simulink model "MIL4L3_SW6_V1_20220211"  (R2018b)
settings: Solver=FixedStepAuto  StartTime=0.0  StopTime=inf  FixedStep=0.001  RelTol=1e-3
PreLoadFcn:
  | A0_MILtest;
undefined symbols (not defined in the file or in its folder): Clb_ICADirect_LaneDisp_StateFive, Clb_ICADirect_LaneDisp_StateFour, Clb_ICADirect_LaneDisp_StateOne, Clb_ICADirect_LaneDisp_StateThree, Clb_ICADirect_LaneDisp_StateTwo, Clb_ICADirect_LaneDisp_StateZero, Clb_ICADirect_LaneDispSW, Clb_ICADirect_TrnLghtsCom_Switch, Clb_ICADirect_TrnLghtsCom_Value, Clb_ICADirect_TrnLghtsCrtl_Inhb, IMAP_Clb_ACU_Driver_Belt, IMAP_Clb_ACU_Driver_Belt_Over, IMAP_Clb_ACU_Passenger_Belt, IMAP_Clb_ACU_Passenger_Belt_Over, IMAP_Clb_ACU_RearLeft_Belt, IMAP_Clb_ACU_RearLeft_Belt_Over, IMAP_Clb_ACU_RearMiddle_Belt, IMAP_Clb_ACU_RearMiddle_Belt_Over, IMAP_Clb_ACU_RearRight_Belt, IMAP_Clb_ACU_RearRight_Belt_Over, IMAP_Clb_AEB_Switch, IMAP_Clb_AEB_Switch_Over, IMAP_Clb_ALC_TLC_Mode, IMAP_Clb_ALC_TLC_Mode_Over, IMAP_Clb_BCM_Battery_Voltage, IMAP_Clb_BCM_Battery_Voltage_Over, IMAP_Clb_BCM_BrakeLamp_State, IMAP_Clb_BCM_BrakeLamp_State_Over, IMAP_Clb_BCM_CHMSL_Status, IMAP_Clb_BCM_CHMSL_Status_Over, IMAP_Clb_BCM_Door_Lock_State, IMAP_Clb_BCM_Door_Lock_State_Over, IMAP_Clb_BCM_FrontWiper_State, IMAP_Clb_BCM_FrontWiper_State_Over, IMAP_Clb_BCM_FrontWiper_Switch, IMAP_Clb_BCM_FrontWiper_Switch_Over, IMAP_Clb_BCM_HazardLamp, IMAP_Clb_BCM_HazardLamp_Over, IMAP_Clb_BCM_HazardLamp_Switch, IMAP_Clb_BCM_HazardLamp_Switch_Over, IMAP_Clb_BCM_HighBeam_State, IMAP_Clb_BCM_HighBeam_State_Over, IMAP_Clb_BCM_Ignition_State, IMAP_Clb_BCM_Ignition_State_Over, IMAP_Clb_BCM_IHBC_Enabled, IMAP_Clb_BCM_IHBC_Enabled_Over, IMAP_Clb_BCM_Left_Light, IMAP_Clb_BCM_Left_Light_Over, IMAP_Clb_BCM_LeftTurn_Switch, IMAP_Clb_BCM_LeftTurn_Switch_Over, IMAP_Clb_BCM_LF_Door_State, IMAP_Clb_BCM_LF_Door_State_Over, IMAP_Clb_BCM_LowBeam_State, IMAP_Clb_BCM_LowBeam_State_Over, IMAP_Clb_BCM_LR_Door_State, IMAP_Clb_BCM_LR_Door_State_Over, IMAP_Clb_BCM_RF_Door_State, IMAP_Clb_BCM_RF_Door_State_Over, IMAP_Clb_BCM_Right_Light, IMAP_Clb_BCM_Right_Light_Over ... (+547)
libraries: CarMaker4SL x2153, simulink x292, dspstat3 x3, canmsglib x2, simulink_extras x1
(part 6 of 52)

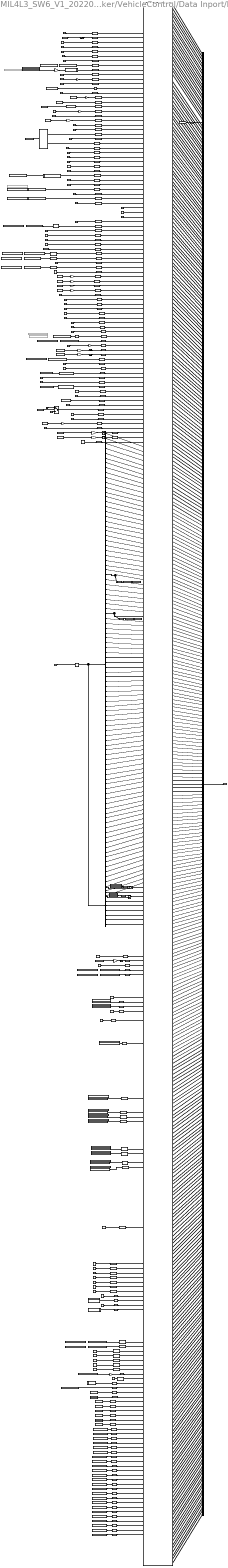
== system MIL4L3_SW6_V1_20220211/CarMaker/VehicleControl/Data Inport/IMAP ==
  note: 根据ACC反馈更新
  note: 需要补充输入数据
  note: 根据规控反馈，由0改为1
  note: 2是打开FAPA
      | else是关闭FAPA
  note: 单位转换：Bar-MPa
  note: 0:无故障
      | 1:故障
  note: 制动轮缸压力
  note: 0：无输入
      | 1：MP5不工作
      | 2：MP5工作
      | 3：无效
  note: 0： Reserved
      | 1： ISA
      | 2： ISLC
      | 3： Reserved
  note: 0：ESA OFF
      | 1：ESA ON
      | 2：Reserved
      | 3： Reserved
  note: 0：Single Lane（ICA）（default）
      | 1：ICAReserved
      | 2：TLC
      | 3：ALC+TLC
  note: 根据规控反馈，由0改为1
  note: 根据acc反馈补充
  note: 0:Available
      | 1:Not available
  note: 0：自适应巡航（ACC）
      | 1：智能领航（ICA）
      | 2：Reserved
      | 3： Reserved
  SDFA_L3- : Inport
  1 : CarMaker4SL/Read CM Dict  xname=Car.vFL  xsync=off
  2 : CarMaker4SL/Read CM Dict  xname=Car.vFR  xsync=off
  3 : CarMaker4SL/Read CM Dict  xname=Car.vRL  xsync=off
  4 : CarMaker4SL/Read CM Dict  xname=Car.vRR  xsync=off
  ACCEL_LONGI_CALIB1 : Saturate  UpperLimit=40.92  LowerLimit=-40.96
  ACU_DriverBeltSwitchSig : Constant  Value=0
  ACU_PassengerBeltSwitchSig : Constant  Value=0
  BCM_BrakeLampStatus : Constant  Value=0
  BCM_CHMSLStatus : Constant  Value=0
  BCM_FrontWiperWorkSt : Constant  Value=0
  BCM_HazardSwitchSt : Constant  Value=0  OutDataTypeStr=uint8
  BCM_HighBeamStatus : Constant  Value=0
  BCM_IgnitionSt : Constant  Value=2
  Bus Selector : BusSelector  OutputSignals=SDFAve_y_ISAValue (signal 28),SDFAve_y_ISAPopupMessage (signal 88),SDFAve_y_ISASignType (signal 86),SDFAve_y_ISAStatus (signal 87),SDFAve_y_TSR_Sign_Type (signal 29),SDFAve_g_CameraSignalFault (signal 30),SDFAve_y_Radar_State (signal 89),SDFAve_y_OperatinfStatus (signal 90),SDFAve_y_Radar_FaultBitSetting_Signal (signal 94)
  Bus Selector1 : BusSelector  OutputSignals=SDFAve_d_sensor_status (signal 1),SDFAve_d_sen_sta_LF_radar (signal 2),SDFAve_d_sen_sta_RF_radar (signal 3),SDFAve_d_sen_sta_LB_radar (signal 4),SDFAve_d_sen_sta_RB_radar (signal 5),SDFAve_d_fusion_status (signal 6),SDFAve_g_fusion_time_stamp (signal 7),SDFAve_d_obj_Num (signal 8),SDFAva_d_obj_id (signal 9),SDFAva_g_obj_pos_x (signal 10),SDFAva_g_obj_pos_y (signal 11),SDFAva_g_obj_vel_x (signal 12),SDFAva_g_obj_vel_y (signal 13),SDFAva_g_obj_acc_x (signal 14),SDFAva_g_obj_acc_y (signal 15),SDFAva_g_obj_pos_var_x (signal 16),SDFAva_g_obj_pos_var_y (signal 17),SDFAva_g_obj_pos_var_xy (signal 18),SDFAva_g_obj_width (signal 19),SDFAva_g_obj_length (signal 20),SDFAva_d_obj_class (signal 21),SDFAva_d_obj_lane (signal 22),SDFAva_y_obj_status (signal 23),SDFAve_g_obj_age (signal 24),SDFAva_y_obj_TurnLight (signal 25),SDFAva_d_obj_BrakeLight (signal 26),SDFAva_y_obj_MotionStatus (signal 27),SDFAve_y_Road_TYPE (signal 31),SDFAve_g_L0_C0_COEF (signal 32),SDFAve_g_L0_C1_COEF (signal 33),SDFAve_g_L0_C2_COEF (signal 34),SDFAve_g_L0_C3_COEF (signal 35),SDFAve_g_L0_VIEW_RANGE (signal 36),SDFAve_g_L0_DETECT_QUALITY (signal 37),SDFAve_d_L0_LINE_TYPE (signal 38),SDFAve_g_L0_MARK_WIDTH (signal 39),SDFAve_g_R0_C0_COEF (signal 40),SDFAve_g_R0_C1_COEF (signal 41),SDFAve_g_R0_C2_COEF (signal 42),SDFAve_g_R0_C3_COEF (signal 43),SDFAve_g_R0_VIEW_RANGE (signal 44),SDFAve_y_R0_DETECT_QUALITY (signal 45),SDFAve_d_R0_LINE_TYPE (signal 46),SDFAve_g_R0_MARK_WIDTH (signal 47),SDFAve_g_R0_VIEW_RANGE (signal 48),SDFAve_g_L1_C1_COEF (signal 49),SDFAve_g_L1_C2_COEF (signal 50),SDFAve_g_L1_C3_COEF (signal 51),SDFAve_g_L1_VIEW_RANGE (signal 52),SDFAve_y_L1_DETECT_QUALITY (signal 53),SDFAve_d_L1_LINE_TYPE (signal 54),SDFAve_g_L1_MARK_WIDTH (signal 55),SDFAve_g_R1_C0_COEF (signal 56),SDFAve_g_R1_C1_COEF (signal 57),SDFAve_g_R1_C2_COEF (signal 58),SDFAve_g_R1_C3_COEF (signal 59),SDFAve_g_R1_VIEW_RANGE (signal 60),SDFAve_y_R1_DETECT_QUALITY (signal 61),SDFAve_d_R1_LINE_TYPE (signal 62),SDFAve_g_R1_MARK_WIDTH (signal 63),SDFAve_g_L0_C0_BACK_COEF (signal 64),SDFAve_g_L0_C1_BACK_COEF (signal 65),SDFAve_g_L0_C2_BACK_COEF (signal 66),SDFAve_g_L0_C3_BACK_COEF (signal 67),SDFAve_g_L0_BACK_RANGE (signal 68),SDFAve_g_R0_C0_BACK_COEF (signal 69),SDFAve_g_R0_C1_BACK_COEF (signal 70),SDFAve_g_L0_C0_BACK_COEF (signal 71),SDFAve_g_R0_C3_BACK_COEF (signal 72),SDFAve_g_R0_BACK_RANGE (signal 73),SDFAve_g_L1_C0_BACK_COEF (signal 74),SDFAve_g_L1_C1_BACK_COEF (signal 75),SDFAve_g_L1_C2_BACK_COEF (signal 76),SDFAve_g_L1_C3_BACK_COEF (signal 77),SDFAve_g_L1_BACK_RANGE (signal 78),SDFAve_g_R1_C0_BACK_COEF (signal 79),SDFAve_g_R1_C1_BACK_COEF (signal 80),SDFAve_g_R1_C2_BACK_COEF (signal 81),SDFAve_g_R1_C3_BACK_COEF (signal 82),SDFAve_g_R1_BACK_RANGE (signal 83),SDFAve_g_Lrg_C0_BACK_COEF (signal 95),SDFAve_g_Lrg_C1_BACK_COEF (signal 96),SDFAve_g_Lrg_C2_BACK_COEF (signal 97),SDFAve_g_Lrg_C3_BACK_COEF (signal 98),SDFAve_g_Lrg_VIEW_RANGE_start (signal 99),SDFAve_g_Lrg_VIEW_RANGE_end (signal 100),SDFAve_y_Lrg_DETECT_QUALITY (signal 109),SDFAve_y_Lrg_LINE_TYPE (signal 110),SDFAve_g_Rrg_C0_BACK_COEF (signal 101),SDFAve_g_Rrg_C1_BACK_COEF (signal 102),SDFAve_g_Rrg_C2_BACK_COEF (signal 103),SDFAve_g_Rrg_C3_BACK_COEF (signal 104),SDFAve_g_Rrg_VIEW_RANGE_start (signal 105),SDFAve_g_Rrg_VIEW_RANGE_end (signal 106),SDFAve_y_Rrg_DETECT_QUALITY (signal 107),SDFAve_y_Rrg_LINE_TYPE (signal 108)
  BusCreator : BusCreator  Inputs=425
  CIPV_ID1 : Subsystem
  Compare To Constant2 : simulink/Logic and Bit Operations/Compare To Constant  relop=>=  const=0.5  OutDataTypeStr=boolean
  Constant{1..2,15,20,22,24..27} (9 alike) : Constant  Value=0
  Constant10 : Constant
  Constant18 : Constant
  Constant19 : Constant
  Constant21 : Constant  Value=2
  Constant23 : Constant  Value=0  OutDataTypeStr=uint8
  Data Type  Conversion{1..16,19..22,24..27,32,36..37,41..42,44..52,54..58,60,63..64,71..73,75..83,86..87,89..96,98..99,101,103..106,108..110,112..113,115,131..134,141,149,156,158..159,162,171,290,292..295,297} (98 alike) : DataTypeConversion
  Data Type  Conversion180 : DataTypeConversion  OutDataTypeStr=UInt16
  Data Type Conversion{,1..13,21..43,46..47,51..54,56,58..59,61,64..65,67,72..73,92,211..212,216,223..227,230,238..241,244,246} (68 alike) : DataTypeConversion
  Data Type Conversion48 : DataTypeConversion  OutDataTypeStr=T_M_Nm_Float32
  Data Type Conversion49 : DataTypeConversion  OutDataTypeStr=T_M_Nm_Float32
  Define CM Dict : CarMaker4SL/Define CM Dict  xname=User.IO.Out.R0_C1  xmono=off  xtype=Double4  xdvaplace=None  xnstates=0  xfirststate=0  xinitial=0
  Define CM Dict1 : CarMaker4SL/Define CM Dict  xname=User.IO.Out.EPS_LKAState  xmono=off  xtype=Double4  xdvaplace=IO_Out  xnstates=0  xfirststate=0  xinitial=0
  Define CM Dict10 : CarMaker4SL/Define CM Dict  xname=User.IO.Out.ISA_SignType  xmono=off  xtype=Double4  xdvaplace=IO_Out  xnstates=0  xfirststate=0  xinitial=0
  Define CM Dict11 : CarMaker4SL/Define CM Dict  xname=User.IO.Out.BCM_LeftTurnSwitchSt  xunit=Nm  xmono=off  xtype=Double4  xdvaplace=IO_Out  xnstates=0  xfirststate=0  xinitial=0
  Define CM Dict12 : CarMaker4SL/Define CM Dict  xname=User.IO.Out.BCM_RightTurnSwicthSt  xunit=Nm  xmono=off  xtype=Double4  xdvaplace=IO_Out  xnstates=0  xfirststate=0  xinitial=0
  Define CM Dict15 : CarMaker4SL/Define CM Dict  Commented=on  xname=User.IO.Out.Brake_pedal_position  xunit=%  xmono=off  xtype=Double4  xdvaplace=IO_Out  xnstates=0  xfirststate=0  xinitial=0
  Define CM Dict17 : CarMaker4SL/Define CM Dict  xname=User.IO.Out.Mp5TLCMode  xunit=Nm  xmono=off  xtype=Double4  xdvaplace=IO_Out  xnstates=0  xfirststate=0  xinitial=0
  Define CM Dict2 : CarMaker4SL/Define CM Dict  xname=User.IO.Out.BCM_HazardLampSt  xmono=off  xtype=Double4  xdvaplace=IO_Out  xnstates=0  xfirststate=0  xinitial=0
  Define CM Dict22 : CarMaker4SL/Define CM Dict  xname=User.IO.Out.EPS_ESAState  xmono=off  xtype=Double4  xdvaplace=IO_Out  xnstates=0  xfirststate=0  xinitial=0
  Define CM Dict27 : CarMaker4SL/Define CM Dict  xname=User.IO.Out.MP5_JA_Modes  xunit=Nm  xmono=off  xtype=Double4  xdvaplace=IO_Out  xnstates=0  xfirststate=0  xinitial=0
  Define CM Dict28 : CarMaker4SL/Define CM Dict  xname=User.IO.Out.MP5_JA_Alert_Switch  xunit=Nm  xmono=off  xtype=Double4  xdvaplace=IO_Out  xnstates=0  xfirststate=0  xinitial=0
  Define CM Dict29 : CarMaker4SL/Define CM Dict  xname=User.IO.Out.MP5_AutoPilotSwitch  xmono=off  xtype=Double4  xdvaplace=IO_Out  xnstates=0  xfirststate=0  xinitial=0
  Define CM Dict3 : CarMaker4SL/Define CM Dict  xname=User.IO.Out.Mp5_ELKSwitch  xunit=Nm  xmono=off  xtype=Double4  xdvaplace=IO_Out  xnstates=0  xfirststate=0  xinitial=0
  Define CM Dict30 : CarMaker4SL/Define CM Dict  xname=User.IO.Out.Mp5_ISAMode  xunit=Nm  xmono=off  xtype=Double4  xdvaplace=IO_Out  xnstates=0  xfirststate=0  xinitial=0
  Define CM Dict32 : CarMaker4SL/Define CM Dict  xname=User.IO.Out.MP5_ESASwitch  xunit=Nm  xmono=off  xtype=Double4  xdvaplace=IO_Out  xnstates=0  xfirststate=0  xinitial=0
  Define CM Dict33 : CarMaker4SL/Define CM Dict  xname=User.IO.Out.EPS_DriverInitializedESA  xunit=Nm  xmono=off  xtype=Double4  xdvaplace=IO_Out  xnstates=0  xfirststate=0  xinitial=0
  Define CM Dict36 : CarMaker4SL/Define CM Dict  Commented=on  xname=User.IO.Out.EPS_SteeringHoldState  xmono=off  xtype=Double4  xdvaplace=IO_Out  xnstates=0  xfirststate=0  xinitial=1
  Define CM Dict37 : CarMaker4SL/Define CM Dict  xname=User.IO.Out.EMS_BrakePedalSignal  xmono=off  xtype=Double4  xdvaplace=IO_Out  xnstates=0  xfirststate=0  xinitial=0
  Define CM Dict4 : CarMaker4SL/Define CM Dict  xname=User.IO.Out.Mp5_ISASwitch  xmono=off  xtype=Double4  xdvaplace=IO_Out  xnstates=0  xfirststate=0  xinitial=0
  Define CM Dict43 : CarMaker4SL/Define CM Dict  xname=User.IO.Out.SCC_LeftSteeringWheelSwitchSig  xmono=off  xtype=Double4  xdvaplace=IO_Out  xnstates=0  xfirststate=0  xinitial=0
  Define CM Dict47 : CarMaker4SL/Define CM Dict  xname=User.IO.Out.BCM_LeftlightSt  xunit=Nm  xmono=off  xtype=Double4  xdvaplace=IO_Out  xnstates=0  xfirststate=0  xinitial=0
  Define CM Dict48 : CarMaker4SL/Define CM Dict  xname=User.IO.Out.BCM_RightlightSt  xunit=Nm  xmono=off  xtype=Double4  xdvaplace=IO_Out  xnstates=0  xfirststate=0  xinitial=0
  Define CM Dict5 : CarMaker4SL/Define CM Dict  xname=User.IO.Out.PEPS_DoorLockReq  xunit=Nm  xmono=off  xtype=Double4  xdvaplace=IO_Out  xnstates=0  xfirststate=0  xinitial=0
  Define CM Dict55 : CarMaker4SL/Define CM Dict  xname=User.IO.Out.MP5_AEBSwitch  xmono=off  xtype=Double4  xdvaplace=IO_Out  xnstates=0  xfirststate=0  xinitial=0
  Define CM Dict56 : CarMaker4SL/Define CM Dict  xname=User.IO.Out.MP5_FCWSwitch  xmono=off  xtype=Double4  xdvaplace=IO_Out  xnstates=0  xfirststate=0  xinitial=0
  Define CM Dict58 : CarMaker4SL/Define CM Dict  xname=User.IO.Out.Mp5_LSSSwitch  xmono=off  xtype=Double4  xdvaplace=IO_Out  xnstates=0  xfirststate=0  xinitial=0
  Define CM Dict59 : CarMaker4SL/Define CM Dict  xname=User.IO.Out.Mp5_LSSMode  xmono=off  xtype=Double4  xdvaplace=IO_Out  xnstates=0  xfirststate=0  xinitial=0
  Define CM Dict6 : CarMaker4SL/Define CM Dict  xname=User.IO.Out.BCM_DoorLockSt  xunit=Nm  xmono=off  xtype=Double4  xdvaplace=IO_Out  xnstates=0  xfirststate=0  xinitial=1
  Define CM Dict63 : CarMaker4SL/Define CM Dict  xname=User.IO.Out.EPS_SteeringTorqueValue  xunit=Nm  xmono=off  xtype=Double4  xdvaplace=IO_Out  xnstates=0  xfirststate=0  xinitial=0.5
  Define CM Dict7 : CarMaker4SL/Define CM Dict  Commented=on  xname=User.IO.Out.GW_Mp5_ISA_Switch  xmono=off  xtype=Double4  xdvaplace=IO_Out  xnstates=0  xfirststate=0  xinitial=0
  Define CM Dict8 : CarMaker4SL/Define CM Dict  xname=User.IO.Out.L0_C1  xmono=off  xtype=Double4  xdvaplace=None  xnstates=0  xfirststate=0  xinitial=0
  Define CM Dict9 : CarMaker4SL/Define CM Dict  xname=User.IO.Out.ISA_Value  xmono=off  xtype=Double4  xdvaplace=IO_Out  xnstates=0  xfirststate=0  xinitial=0
  EMS_ACCFunctionIhibition : Constant  Value=0
  EMS_ACCcontrolGearAvailable : Constant
  EMS_ACCcontrolTorqueAvailable : Constant  Value=0
  EMS_AccPedalPos : Constant  Value=0
  EMS_DriverTorque : Constant  Value=0
  EMS_EngRunningStatus : Constant  Value=3
  EMS_HighestGearMinTorque : Constant  Value=0
  EMS_LowerestGearMaxTorque : Constant  Value=0
  EMS_NotControlableMaxPowertra : Constant  Value=0
  EMS_NotControlableMinPowertra : Constant  Value=0
  EPS_DriverOverride : Constant  Value=0
  EPS_SteeringAngle_Flag : Constant
  EPS_TorqueLimitationState : Constant  Value=0
  EPS_WarmingLampSt : Constant  Value=0
  ESC_ABSAlarmSig : Constant  Value=0
  ESC_ABSAlarmSig1 : Constant  Value=0
  ESC_ABSValidity1 : Constant  Value=0
  ESC_ABSWorkLable : Constant  Value=0
  ESC_BrakeReleasedFailsafe : Constant  Value=0
  ESC_BrakingEffort : Constant  Value=0
  ESC_DynamicSlope : Constant  Value=0
  ESC_DynamicSlopeAccuracy : Constant  Value=0
  ESC_EPBStaus : Constant  Value=0  OutDataTypeStr=Inherit: Inherit via back propagation
  ESC_ESCOFF : Constant  Value=0
  ESC_ESCWorkStatus : Constant  Value=0
  ESC_FLWHeelPulseCounter : Constant  Value=0
  ESC_FLWHeelPulseCounterValidity : Constant  Value=0
  ESC_FLWHeelSpdFaultSignal1 : Constant  Value=0
  ESC_FRWHeelPulseCounter : Constant  Value=0
  ESC_FRWHeelSpdFaultSignal1 : Constant  Value=0
  ESC_LateralAccelaration : CarMaker4SL/Read CM Dict  xname=Car.ay  xsync=off
  ESC_LongitudinalAccelervalidity : Constant  Value=0
  ESC_RLWHeelPulseCounter : Constant  Value=0
  ESC_RLWHeelPulseCounterValidity : Constant  Value=0
  ESC_RLWHeelSpdFaultSignal1 : Constant  Value=0
  ESC_RRWHeelPulseCounter : Constant  Value=0
  ESC_RRWHeelPulseCounterValidity : Constant  Value=0
  ESC_RRWHeelSpdFaultSignal1 : Constant  Value=0
  ESC_Static_slope : Constant  Value=0
  ESC_TCSCtlActive : Constant
  ESC_VehDrivingDirection : Constant
  ESC_VehSpdValidFlag : Constant  Value=0
  ESC_VehicleHoldStatus : Constant  Value=0
  Front_right_pulse_malfunction : Constant  Value=0
  GW_SCC_RightSteeringWheelSwitch : Constant  Value=0
  GW_TCU_DCTClutchStatus : Constant  Value=0
  Gain : Gain  Gain=1/100
  Gain1 : Gain  Gain=180/pi
  Gain{9..12} (4 alike) : Gain  Gain=100
  Gain15 : Gain  Gain=180/pi
  Gain16 : Gain  Gain=0.1
  Gain17 : Gain  Gain=180/pi  OutDataTypeStr=T_M_Nm_Float32
  Gain{2,4..7} (5 alike) : Gain  Gain=3.6
  Gain25 : Gain  Gain=180/pi  OutDataTypeStr=T_M_Nm_Float32
  Gain3 : Gain  Gain=180/pi
  Gain8 : Gain  Gain=30/pi
  IC_TotalOdemeter : Constant  Value=0
  MP5_FCWSensitivity : Constant  Value=0
  MP5_HazardLampCtrlReq : Constant  Value=0  OutDataTypeStr=uint8
  MSRinRegulation : Constant  Value=0
  Manual Switch1 : ManualSwitch
  Manual Switch2 : ManualSwitch
  Mp5_TSRSwitch : Constant  Value=0
  Rate Transition : RateTransition  OutPortSampleTime=0.001
  Read CM Dict : CarMaker4SL/Read CM Dict  xname=User.IO.Out.IFC_Line01_CurvChange  xsync=off
  Read CM Dict1 : CarMaker4SL/Read CM Dict  xname=User.IO.Out.EPS_LKAState  xsync=off
  Read CM Dict10 : CarMaker4SL/Read CM Dict  xname=PT.Engine.Trq  xsync=off
  Read CM Dict11 : CarMaker4SL/Read CM Dict  xname=PT.Engine.Trq  xsync=off
  Read CM Dict12 : CarMaker4SL/Read CM Dict  xname=User.IO.Out.BCM_DoorLockSt  xsync=off
  Read CM Dict13 : CarMaker4SL/Read CM Dict  xname=User.IO.Out.BCM_LeftTurnSwitchSt  xsync=off
  Read CM Dict14 : CarMaker4SL/Read CM Dict  xname=Car.v  xsync=off
  Read CM Dict15 : CarMaker4SL/Read CM Dict  xname=User.IO.Out.BCM_RightTurnSwicthSt  xsync=off
  Read CM Dict16 : CarMaker4SL/Read CM Dict  xname=PT.Engine.rotv  xsync=off
  Read CM Dict17 : CarMaker4SL/Read CM Dict  xname=PT.TCU.GB.GearNoTrg  xsync=off
  Read CM Dict18 : CarMaker4SL/Read CM Dict  xname=User.IO.Out.ISA_Value  xsync=off
  Read CM Dict19 : CarMaker4SL/Read CM Dict  xname=Steer.WhlVel  xsync=off
  Read CM Dict2 : CarMaker4SL/Read CM Dict  xname=User.IO.Out.Mp5_ELKSwitch  xsync=off
  Read CM Dict20 : CarMaker4SL/Read CM Dict  xname=Steer.WhlAng  xsync=off
  Read CM Dict21 : CarMaker4SL/Read CM Dict  Commented=on  xname=User.IO.Out.EPS_SteeringHoldState  xsync=off
  Read CM Dict22 : CarMaker4SL/Read CM Dict  xname=User.IO.Out.Mp5_ISASwitch  xsync=off
  Read CM Dict23 : CarMaker4SL/Read CM Dict  xname=Brake.Hyd.Sys.pMC  xsync=off
  Read CM Dict24 : CarMaker4SL/Read CM Dict  xname=Car.ax  xsync=off
  Read CM Dict25 : CarMaker4SL/Read CM Dict  xname=User.IO.Out.ISA_SignType  xsync=off
  Read CM Dict26 : CarMaker4SL/Read CM Dict  xname=DM.Gas  xsync=off
  Read CM Dict27 : CarMaker4SL/Read CM Dict  xname=User.IO.Out.MP5_AEBSwitch  xsync=off
  Read CM Dict28 : CarMaker4SL/Read CM Dict  xname=PT.GearBox.GearNo  xsync=off
  Read CM Dict29 : CarMaker4SL/Read CM Dict  xname=User.IO.Out.Mp5_LSSSwitch  xsync=off
  Read CM Dict3 : CarMaker4SL/Read CM Dict  xname=User.IO.Out.EMS_BrakePedalSignal  xsync=off
  Read CM Dict30 : CarMaker4SL/Read CM Dict  xname=User.IO.Out.Mp5_LSSMode  xsync=off
  Read CM Dict31 : CarMaker4SL/Read CM Dict  xname=User.IO.Out.MP5_FCWSwitch  xsync=off
  Read CM Dict32 : CarMaker4SL/Read CM Dict  xname=User.IO.Out.EPS_SteeringTorqueValue  xsync=off
  Read CM Dict33 : CarMaker4SL/Read CM Dict  xname=User.IO.Out.IFC_Line01_Dy  xsync=off
  Read CM Dict34 : CarMaker4SL/Read CM Dict  xname=User.IO.Out.VR_R1  xsync=off
  Read CM Dict35 : CarMaker4SL/Read CM Dict  xname=User.IO.Out.VR_R0  xsync=off
  Read CM Dict36 : CarMaker4SL/Read CM Dict  xname=User.IO.Out.EPS_SteeringTorqueValue  xsync=off
  Read CM Dict4 : CarMaker4SL/Read CM Dict  xname=User.IO.Out.SCC_LeftSteeringWheelSwitchSig  xsync=off
  Read CM Dict41 : CarMaker4SL/Read CM Dict  xname=User.IO.Out.IFC_Line01_Type  xsync=off
  Read CM Dict42 : CarMaker4SL/Read CM Dict  xname=User.IO.Out.VR_L1  xsync=off
  Read CM Dict43 : CarMaker4SL/Read CM Dict  xname=User.IO.Out.VR_L0  xsync=off
  Read CM Dict44 : CarMaker4SL/Read CM Dict  xname=User.IO.Out.EPS_DriverInitializedESA  xsync=off
  Read CM Dict48 : CarMaker4SL/Read CM Dict  xname=User.IO.Out.IFC_Line02_CurvChange  xsync=off
  Read CM Dict49 : CarMaker4SL/Read CM Dict  xname=User.IO.Out.IFC_Line02_Curv  xsync=off
  Read CM Dict5 : CarMaker4SL/Read CM Dict  xname=DM.Gas  xsync=off
  Read CM Dict50 : CarMaker4SL/Read CM Dict  xname=User.IO.Out.IFC_Line02_HeadingAngle  xsync=off
  Read CM Dict51 : CarMaker4SL/Read CM Dict  xname=User.IO.Out.IFC_Line02_Dy  xsync=off
  Read CM Dict53 : CarMaker4SL/Read CM Dict  xname=Car.YawRate  xsync=off
  Read CM Dict54 : CarMaker4SL/Read CM Dict  xname=User.IO.Out.IFC_Line02_Type  xsync=off
  Read CM Dict6 : CarMaker4SL/Read CM Dict  xname=Car.v  xsync=off
  Read CM Dict61 : CarMaker4SL/Read CM Dict  xname=User.IO.Out.IFC_Line03_CurvChange  xsync=off
  Read CM Dict62 : CarMaker4SL/Read CM Dict  xname=User.IO.Out.IFC_Line03_Curv  xsync=off
  Read CM Dict63 : CarMaker4SL/Read CM Dict  xname=User.IO.Out.IFC_Line03_HeadingAngle  xsync=off
  Read CM Dict64 : CarMaker4SL/Read CM Dict  xname=User.IO.Out.IFC_Line03_Dy  xsync=off
  Read CM Dict67 : CarMaker4SL/Read CM Dict  xname=User.IO.Out.IFC_Line03_Type  xsync=off
  Read CM Dict69 : CarMaker4SL/Read CM Dict  xname=User.IO.Out.EPS_ESAState  xsync=off
  Read CM Dict7 : CarMaker4SL/Read CM Dict  xname=User.IO.Out.BCM_HazardLampSt  xsync=off
  Read CM Dict71 : CarMaker4SL/Read CM Dict  xname=Steer.WhlAng  xsync=off
  Read CM Dict73 : CarMaker4SL/Read CM Dict  xname=User.IO.Out.BCM_LeftlightSt  xsync=off
  Read CM Dict74 : CarMaker4SL/Read CM Dict  xname=User.IO.Out.IFC_Line04_CurvChange  xsync=off
  Read CM Dict75 : CarMaker4SL/Read CM Dict  xname=User.IO.Out.IFC_Line04_Curv  xsync=off
  Read CM Dict76 : CarMaker4SL/Read CM Dict  xname=User.IO.Out.IFC_Line04_HeadingAngle  xsync=off
  Read CM Dict77 : CarMaker4SL/Read CM Dict  xname=User.IO.Out.IFC_Line04_Dy  xsync=off
  Read CM Dict79 : CarMaker4SL/Read CM Dict  xname=User.IO.Out.BCM_RightlightSt  xsync=off
  Read CM Dict8 : CarMaker4SL/Read CM Dict  xname=User.IO.Out.PEPS_DoorLockReq  xsync=off
  Read CM Dict80 : CarMaker4SL/Read CM Dict  xname=User.IO.Out.IFC_Line04_Type  xsync=off
  Read CM Dict81 : CarMaker4SL/Read CM Dict  xname=User.IO.Out.Mp5TLCMode  xsync=off
  Read CM Dict83 : CarMaker4SL/Read CM Dict  xname=User.IO.Out.MP5_JA_Modes  xsync=off
  Read CM Dict84 : CarMaker4SL/Read CM Dict  xname=User.IO.Out.MP5_JA_Alert_Switch  xsync=off
  Read CM Dict85 : CarMaker4SL/Read CM Dict  xname=User.IO.Out.MP5_AutoPilotSwitch  xsync=off
  Read CM Dict86 : CarMaker4SL/Read CM Dict  xname=User.IO.Out.Mp5_ISAMode  xsync=off
  Read CM Dict87 : CarMaker4SL/Read CM Dict  xname=User.IO.Out.ObjCount  xsync=off
  Read CM Dict88 : CarMaker4SL/Read CM Dict  xname=User.IO.Out.IFC_Line01_Curv  xsync=off
  Read CM Dict89 : CarMaker4SL/Read CM Dict  xname=User.IO.Out.IFC_Line01_HeadingAngle  xsync=off
  Read CM Dict9 : CarMaker4SL/Read CM Dict  xname=PT.GearBox.GearNo  xsync=off
  Read CM Dict90 : CarMaker4SL/Read CM Dict  xname=User.IO.Out.MP5_ESASwitch  xsync=off
  Read CM Dict92 : CarMaker4SL/Read CM Dict  xname=Brake.Hyd.Sys.pWB_FL  xsync=off
  Read CM Dict96 : CarMaker4SL/Read CM Dict  xname=Car.YawRate  xsync=off
  Runnable_IMAP_10ms_sys : Subsystem  TreatAsAtomicUnit=on
  SAS_CalibratedStatus : Constant
  SAS_SASFailureSts : Constant
  SAS_TrimmingStatus : Constant
  Saturation : Saturate  UpperLimit=1016  LowerLimit=0
  Saturation1 : Saturate  UpperLimit=780  LowerLimit=-780
  Saturation5 : Saturate  UpperLimit=780  LowerLimit=-780
  Subsystem11 : Subsystem
  Subsystem15 : Subsystem
  Subsystem16 : Subsystem
  Subsystem160 : Subsystem
  Subsystem17 : Subsystem
  Subsystem18 : Subsystem
  Subsystem19 : Subsystem
  Subsystem192 : Subsystem
  Subsystem2 : Subsystem
  Subsystem203 : Subsystem
  Subsystem204 : Subsystem
  Subsystem208 : Subsystem
  Subsystem21 : Subsystem
  Subsystem210 : Subsystem
  Subsystem223 : Subsystem
  Subsystem228 : Subsystem
  Subsystem24 : Subsystem
  Switch : Switch  Criteria=u2 > Threshold  Threshold=0.1
  TBOX_RemoteHazardReq : Constant  Value=0  OutDataTypeStr=uint8
  TCU_ATFailure : Constant  Value=0
  TCU_GearEngagement : Constant
  TCU_SelectedATMode : Constant  Value=0
  Write CM Dict : CarMaker4SL/Write CM Dict  xname=User.IO.Out.R0_C1  xsync=off
  Write CM Dict1 : CarMaker4SL/Write CM Dict  xname=User.IO.Out.L0_C1  xsync=off
  Yaw_speed3 : Saturate  UpperLimit=100  LowerLimit=-100  OutDataTypeStr=T_M_Nm_Float32
  Yaw_speed4 : Saturate  UpperLimit=163.68  LowerLimit=-163.84  OutDataTypeStr=T_M_Nm_Float32
  IMAP_Output : Outport
  wires:
  Data Type Conversion212/1 -> Runnable_IMAP_10ms_sys/314(SDFAve_g_ORI_L1_C0)  "IFC_Line03_Dy"
  Data Type Conversion21/1 -> Runnable_IMAP_10ms_sys/294(FAPAve_Cnt_AdvancedParkingAssist)  "Cnt_AdvancedParkingAssist"
  Constant15/1 -> Data Type Conversion21/1
  Data Type Conversion64/1 -> Runnable_IMAP_10ms_sys/296(SDFAve_d_ORI_Obj_Num)  "IFC_ObjHdr_ObjCount"
  Data Type Conversion53/1 -> Runnable_IMAP_10ms_sys/297(SDFAva_d_ORI_Obj_Class)  "IFC_obj_Type"
  Read CM Dict62/1 -> Data Type Conversion73/1
  Read CM Dict63/1 -> Data Type Conversion211/1
  Read CM Dict88/1 -> Data Type Conversion58/1
  Read CM Dict49/1 -> Data Type Conversion225/1
  Read CM Dict48/1 -> Data Type Conversion223/1
  Read CM Dict87/1 -> Data Type Conversion64/1
  Data Type Conversion58/1 -> Runnable_IMAP_10ms_sys/306(SDFAve_g_ORI_L0_C2)  "IFC_Line01_Curv"
  Read CM Dict54/1 -> Data Type Conversion230/1
  Read CM Dict61/1 -> Data Type Conversion72/1
  Data Type Conversion56/1 -> Runnable_IMAP_10ms_sys/305(SDFAve_g_ORI_L0_C3)  "IFC_Line01_CurvChange"
  Data Type Conversion27/1 -> Runnable_IMAP_10ms_sys/310(SDFAve_g_ORI_L0_VR)  "VR_L0"
  Subsystem228/1(obj_Type) -> Data Type Conversion53/1
  Data Type Conversion59/1 -> Runnable_IMAP_10ms_sys/307(SDFAve_g_ORI_L0_C1)  "IFC_Line01_HeadingAngle"
  Read CM Dict80/1 -> Data Type Conversion244/1
  Data Type Conversion211/1 -> Runnable_IMAP_10ms_sys/313(SDFAve_g_ORI_L1_C1)  "IFC_Line03_HeadingAngle"
  Data Type Conversion73/1 -> Runnable_IMAP_10ms_sys/312(SDFAve_g_ORI_L1_C2)  "IFC_Line03_Curv"
  Read CM Dict77/1 -> Data Type Conversion241/1
  Read CM Dict67/1 -> Data Type Conversion216/1
  Subsystem223/1(obj_ID) -> Data Type Conversion51/1
  Read CM Dict64/1 -> Data Type Conversion212/1
  Read CM Dict/1 -> Data Type Conversion56/1
  Read CM Dict89/1 -> Data Type Conversion59/1
  Read CM Dict74/1 -> Data Type Conversion238/1
  Read CM Dict76/1 -> Data Type Conversion240/1
  Read CM Dict33/1 -> Data Type Conversion61/1
  Data Type Conversion51/1 -> Runnable_IMAP_10ms_sys/298(SDFAva_d_ORI_Obj_ID)  "IFC_obj_ID"
  Read CM Dict75/1 -> Data Type Conversion239/1
  Data Type Conversion65/1 -> Runnable_IMAP_10ms_sys/309(SDFAve_d_ORI_L0_Type)  "IFC_Line01_Type"
  Read CM Dict51/1 -> Data Type Conversion227/1
  Read CM Dict50/1 -> Data Type Conversion226/1
  CIPV_ID1/1(Out1) -> Data Type Conversion46/1  "CIVP_ID"
  Data Type Conversion46/1 -> Runnable_IMAP_10ms_sys/295(SDFAve_d_ORI_CIPV_ID)  "IFC_VD_CIPV_ID"
  Data Type Conversion61/1 -> Runnable_IMAP_10ms_sys/308(SDFAve_g_ORI_L0_C0)  "IFC_Line01_Dy"
  Data Type Conversion72/1 -> Runnable_IMAP_10ms_sys/311(SDFAve_g_ORI_L1_C3)  "IFC_Line03_CurvChange"
  Read CM Dict41/1 -> Data Type Conversion65/1
  Read CM Dict34/1 -> Data Type Conversion23/1
  Read CM Dict35/1 -> Data Type Conversion25/1
  Read CM Dict42/1 -> Data Type Conversion26/1
  Read CM Dict43/1 -> Data Type Conversion27/1
  Read CM Dict53/1 -> Gain25/1  "ESC_UnfileedYawRate"
  Yaw_speed4/1 -> Data Type Conversion49/1
  Constant26/1 -> Data Type Conversion28/1
  Data Type Conversion29/1 -> Runnable_IMAP_10ms_sys/292(SWINve_y_BCM_LRDoorSwitchSt)  "BCM_LRDoorSwitchSt"
  Data Type Conversion22/1 -> Runnable_IMAP_10ms_sys/286(SWINve_y_BCM_LeftlightSt)  "BCMLeftLightSt"
  ESC_RRWHeelSpdFaultSignal1/1 -> Data Type  Conversion134/1
  Data Type  Conversion6/1 -> Runnable_IMAP_10ms_sys/271(SWINve_y_ESC_ABSAlarmSig)  "ESC_ABSAlarmSig"
  Read CM Dict79/1 -> Data Type Conversion34/1  "BCMRightLightSt"
  Data Type Conversion36/1 -> Runnable_IMAP_10ms_sys/233(SWINve_y_Mp5_ISAMode)  "Mp5_ISAMode"
  Data Type  Conversion149/1 -> Runnable_IMAP_10ms_sys/206(SWINve_y_EPS_ESAState)  "EPS_ESAState"
  ESC_RLWHeelSpdFaultSignal1/1 -> Data Type  Conversion133/1
  Read CM Dict90/1 -> Data Type Conversion38/1
  Data Type  Conversion4/1 -> Runnable_IMAP_10ms_sys/269(SWINve_y_ESC_LongitudinalAccelervalidity)  "ESC_LongitudinalAccelervalidity"
  Gain15/1 -> Saturation5/1
  Read CM Dict73/1 -> Data Type Conversion22/1  "BCMLeftLightSt"
  Read CM Dict81/1 -> Data Type Conversion32/1  "MP5_TLCModeSelection"
  Bus Selector1/7 -> Runnable_IMAP_10ms_sys/97(SDFAve_d_fusion_time_stamp)  "<SDFAve_g_fusion_time_stamp (signal 7)>"
  Data Type Conversion43/1 -> Runnable_IMAP_10ms_sys/293(SWINve_g_ESC_BrakeWheelCylinderPressure)  "ESC_BrakeWheelCylinderPressure"
  Data Type Conversion34/1 -> Runnable_IMAP_10ms_sys/287(SWINve_y_BCM_RightlightSt)  "BCMRightLightSt"
  Read CM Dict71/1 -> Gain15/1  "EPS_SteeringAngle"
  Read CM Dict86/1 -> Data Type Conversion36/1
  Saturation5/1 -> Data Type  Conversion141/1
  Constant27/1 -> Data Type Conversion29/1
  SDFA_L3-/1 -> Rate Transition/1
  Read CM Dict84/1 -> Data Type Conversion42/1
  Data Type Conversion39/1 -> Runnable_IMAP_10ms_sys/244(SWINve_y_MP5_JA_Modes)  "MP5_JA_Modes"
  Read CM Dict92/1 -> Gain16/1  "ESC_BrakeWheelCylinderPressure"
  Data Type  Conversion162/1 -> Runnable_IMAP_10ms_sys/270(SWINve_y_ESC_ABSValidity)  "ESC_ABSValidity"
  Rate Transition/1 -> Bus Selector/1, Bus Selector1/1
  Gain17/1 -> Yaw_speed3/1
  Read CM Dict83/1 -> Data Type Conversion39/1
  Bus Selector1/2 -> Runnable_IMAP_10ms_sys/92(SDFAve_d_sen_sta_LF_radar)  "<SDFAve_d_sen_sta_LF_radar (signal 2)>"
  Bus Selector1/20 -> Runnable_IMAP_10ms_sys/110(SDFAva_g_obj_length)  "<SDFAva_g_obj_length (signal 20)>"
  Bus Selector1/6 -> Runnable_IMAP_10ms_sys/96(SDFAve_d_fusion_status)  "<SDFAve_d_fusion_status (signal 6)>"
  Bus Selector1/24 -> Runnable_IMAP_10ms_sys/114(SDFAva_d_obj_age)  "<SDFAve_g_obj_age (signal 24)>"
  Bus Selector1/17 -> Runnable_IMAP_10ms_sys/107(SDFAva_g_obj_pos_var_y)  "<SDFAva_g_obj_pos_var_y (signal 17)>"
  Bus Selector1/22 -> Runnable_IMAP_10ms_sys/112(SDFAva_y_obj_lane)  "<SDFAva_d_obj_lane (signal 22)>"
  Bus Selector1/26 -> Runnable_IMAP_10ms_sys/116(SDFAva_y_obj_BrakeLight)  "<SDFAva_d_obj_BrakeLight (signal 26)>"
  Bus Selector1/14 -> Runnable_IMAP_10ms_sys/104(SDFAva_g_obj_acc_x)  "<SDFAva_g_obj_acc_x (signal 14)>"
  Bus Selector1/3 -> Runnable_IMAP_10ms_sys/93(SDFAve_d_sen_sta_RF_radar)  "<SDFAve_d_sen_sta_RF_radar (signal 3)>"
  Bus Selector1/15 -> Runnable_IMAP_10ms_sys/105(SDFAva_g_obj_acc_y)  "<SDFAva_g_obj_acc_y (signal 15)>"
  Data Type Conversion49/1 -> Runnable_IMAP_10ms_sys/89(SWINve_g_ESC_UnfilteredYawRate)  "ESC_UnfilteredYawRate"
  Constant21/1 -> Data Type  Conversion158/1
  Bus Selector1/13 -> Runnable_IMAP_10ms_sys/103(SDFAva_g_obj_vel_y)  "<SDFAva_g_obj_vel_y (signal 13)>"
  Yaw_speed3/1 -> Data Type Conversion48/1  "ESC_YawRate"
  Data Type  Conversion131/1 -> Runnable_IMAP_10ms_sys/272(SWINve_y_ESC_FLWHeelSpdFaultSignal)  "ESC_FLWHeelSpdFaultSignal"
  Gain25/1 -> Yaw_speed4/1
  Data Type Conversion32/1 -> Runnable_IMAP_10ms_sys/236(SWINve_y_MP5_TLCModeSelection)  "MP5_TLCModeSelection"
  Bus Selector1/12 -> Runnable_IMAP_10ms_sys/102(SDFAva_g_obj_vel_x)  "<SDFAva_g_obj_vel_x (signal 12)>"
  Data Type Conversion41/1 -> Runnable_IMAP_10ms_sys/278(SWINve_y_ESC_ACCAvailable)  "ESC_ACCAvailable"
  ESC_FLWHeelSpdFaultSignal1/1 -> Data Type  Conversion131/1
  Data Type  Conversion158/1 -> Runnable_IMAP_10ms_sys/216(SWINve_y_MP5_WorkSt)  "MP5_WorkSt"
  Bus Selector1/8 -> Runnable_IMAP_10ms_sys/98(SDFAve_d_obj_Num)  "<SDFAve_d_obj_Num (signal 8)>"
  Bus Selector1/9 -> Runnable_IMAP_10ms_sys/99(SDFAva_y_obj_id)  "<SDFAva_d_obj_id (signal 9)>"
  ESC_FRWHeelSpdFaultSignal1/1 -> Data Type  Conversion132/1
  Constant20/1 -> Data Type Conversion47/1
  Gain16/1 -> Data Type Conversion43/1  "ESC_BrakeWheelCylinderPressure"
  Bus Selector1/23 -> Runnable_IMAP_10ms_sys/113(SDFAva_d_obj_status)  "<SDFAva_y_obj_status (signal 23)>"
  Data Type Conversion48/1 -> Runnable_IMAP_10ms_sys/88(SWINve_g_ESC_YawRate)  "ESC_YawRate"
  Data Type Conversion40/1 -> Runnable_IMAP_10ms_sys/276(SWINve_y_ESC_AEBAvailable)  "ESC_AEBAvailable"
  Data Type Conversion28/1 -> Runnable_IMAP_10ms_sys/291(SWINve_y_BCM_RRDoorSwitchSt)  "BCM_RRDoorSwitchSt"
  Data Type  Conversion171/1 -> Runnable_IMAP_10ms_sys/205(SWINve_y_EPS_DriverInitializedESA)  "EPS_DriverInitializedESA"
  Read CM Dict69/1 -> Data Type  Conversion149/1
  Data Type  Conversion141/1 -> Runnable_IMAP_10ms_sys/203(SWINve_g_EPS_SteeringAngle)  "EPS_SteeringAngle"
  Constant18/1 -> Data Type Conversion40/1  "ESC_AEBAvailable"
  Data Type Conversion47/1 -> Runnable_IMAP_10ms_sys/288(SWINve_y_BCM_TrunkSt)  "BCM_TrunkSt"
  Bus Selector1/1 -> Runnable_IMAP_10ms_sys/91(SDFAve_d_sensor_status)  "<SDFAve_d_sensor_status (signal 1)>"
  Constant19/1 -> Data Type Conversion41/1  "ESC_ACCAvailable"
  Constant25/1 -> Data Type Conversion54/1
  Data Type Conversion52/1 -> Runnable_IMAP_10ms_sys/289(SWINve_y_BCM_LFDoorSwitchSt)  "BCM_LFDoorSwitchSt"
  Constant24/1 -> Data Type Conversion52/1
  Read CM Dict96/1 -> Gain17/1  "ESC_YawRate"
  Bus Selector1/11 -> Runnable_IMAP_10ms_sys/101(SDFAva_g_obj_pos_y)  "<SDFAva_g_obj_pos_y (signal 11)>"
  Data Type  Conversion156/1 -> Runnable_IMAP_10ms_sys/204(SWINve_y_EPS_DriverOverride)  "EPS_DriverOverride"
  Bus Selector1/5 -> Runnable_IMAP_10ms_sys/95(SDFAve_d_sen_sta_RB_radar)  "<SDFAve_d_sen_sta_RB_radar (signal 5)>"
  Bus Selector1/27 -> Runnable_IMAP_10ms_sys/117(SDFAva_y_obj_MotionStatus)  "<SDFAva_y_obj_MotionStatus (signal 27)>"
  Read CM Dict44/1 -> Data Type  Conversion171/1
  Subsystem2/1(ESC_AEBActive) -> Data Type Conversion30/1  "ESC_AEBActive"
  Data Type Conversion54/1 -> Runnable_IMAP_10ms_sys/290(SWINve_y_BCM_RFDoorSwitchSt)  "BCM_RFDoorSwitchSt"
  EPS_DriverOverride/1 -> Data Type  Conversion156/1  "EPS_DriverOverride"
  Subsystem11/1(IMAPve_d_ESC_ACC_Active) -> Data Type Conversion31/1  "ESC_ACCActive"
  Data Type  Conversion132/1 -> Runnable_IMAP_10ms_sys/273(SWINve_y_ESC_FRWHeelSpdFaultSignal)  "ESC_FRWHeelSpdFaultSignal"
  Constant22/1 -> Data Type  Conversion180/1  "System_Clock"
  Data Type Conversion30/1 -> Runnable_IMAP_10ms_sys/277(SWINve_y_ESC_AEBActive)  "ESC_AEBActive"
  Bus Selector1/4 -> Runnable_IMAP_10ms_sys/94(SDFAve_d_sen_sta_LB_radar)  "<SDFAve_d_sen_sta_LB_radar (signal 4)>"
  EPS_SteeringAngle_Flag/1 -> Data Type  Conversion32/1  "EPS_SteeringAngle_Flag"
  ESC_ABSValidity1/1 -> Data Type  Conversion162/1  "ESC_ABSValidity"
  Bus Selector1/19 -> Runnable_IMAP_10ms_sys/109(SDFAva_g_obj_width)  "<SDFAva_g_obj_width (signal 19)>"
  Bus Selector1/16 -> Runnable_IMAP_10ms_sys/106(SDFAva_g_obj_pos_var_x)  "<SDFAva_g_obj_pos_var_x (signal 16)>"
  Bus Selector1/10 -> Runnable_IMAP_10ms_sys/100(SDFAva_g_obj_pos_x)  "<SDFAva_g_obj_pos_x (signal 10)>"
  Bus Selector1/21 -> Runnable_IMAP_10ms_sys/111(SDFAva_y_obj_class)  "<SDFAva_d_obj_class (signal 21)>"
  Bus Selector1/18 -> Runnable_IMAP_10ms_sys/108(SDFAva_g_obj_pos_var_xy)  "<SDFAva_g_obj_pos_var_xy (signal 18)>"
  Data Type  Conversion180/1 -> Runnable_IMAP_10ms_sys/90(System_Clock)
  Bus Selector1/25 -> Runnable_IMAP_10ms_sys/115(SDFAva_y_obj_TurnLight)  "<SDFAva_y_obj_TurnLight (signal 25)>"
  Bus Selector1/28 -> Runnable_IMAP_10ms_sys/118(SDFAve_y_ROAD_TYPE)  "<SDFAve_y_Road_TYPE (signal 31)>"
  Bus Selector1/29 -> Runnable_IMAP_10ms_sys/119(SDFAve_g_L0_C0_COEF)  "<SDFAve_g_L0_C0_COEF (signal 32)>"
  Bus Selector1/30 -> Runnable_IMAP_10ms_sys/120(SDFAve_g_L0_C1_COEF), Data Type Conversion5/1  "<SDFAve_g_L0_C1_COEF (signal 33)>"
  Bus Selector1/31 -> Runnable_IMAP_10ms_sys/121(SDFAve_g_L0_C2_COEF)  "<SDFAve_g_L0_C2_COEF (signal 34)>"
  Bus Selector1/32 -> Runnable_IMAP_10ms_sys/122(SDFAve_g_L0_C3_COEF)  "<SDFAve_g_L0_C3_COEF (signal 35)>"
  Bus Selector1/33 -> Runnable_IMAP_10ms_sys/123(SDFAve_g_L0_VIEW_RANGE)  "<SDFAve_g_L0_VIEW_RANGE (signal 36)>"
  Bus Selector1/34 -> Runnable_IMAP_10ms_sys/124(SDFAve_y_L0_DETECT_QUALITY)  "<SDFAve_g_L0_DETECT_QUALITY (signal 37)>"
  Bus Selector1/35 -> Runnable_IMAP_10ms_sys/125(SDFAve_d_L0_LINE_TYPE)  "<SDFAve_d_L0_LINE_TYPE (signal 38)>"
  Bus Selector1/36 -> Runnable_IMAP_10ms_sys/126(SDFAve_g_L0_MARK_WIDTH)  "<SDFAve_g_L0_MARK_WIDTH (signal 39)>"
  Bus Selector1/37 -> Runnable_IMAP_10ms_sys/127(SDFAve_g_R0_C0_COEF)  "<SDFAve_g_R0_C0_COEF (signal 40)>"
  Bus Selector1/38 -> Runnable_IMAP_10ms_sys/128(SDFAve_g_R0_C1_COEF), Data Type Conversion6/1  "<SDFAve_g_R0_C1_COEF (signal 41)>"
  Bus Selector1/39 -> Runnable_IMAP_10ms_sys/129(SDFAve_g_R0_C2_COEF)  "<SDFAve_g_R0_C2_COEF (signal 42)>"
  Bus Selector1/40 -> Runnable_IMAP_10ms_sys/130(SDFAve_g_R0_C3_COEF)  "<SDFAve_g_R0_C3_COEF (signal 43)>"
  Bus Selector1/41 -> Runnable_IMAP_10ms_sys/131(SDFAve_g_R0_VIEW_RANGE)  "<SDFAve_g_R0_VIEW_RANGE (signal 44)>"
  Bus Selector1/42 -> Runnable_IMAP_10ms_sys/132(SDFAve_y_R0_DETECT_QUALITY)  "<SDFAve_y_R0_DETECT_QUALITY (signal 45)>"
  Bus Selector1/43 -> Runnable_IMAP_10ms_sys/133(SDFAve_d_R0_LINE_TYPE)  "<SDFAve_d_R0_LINE_TYPE (signal 46)>"
  Bus Selector1/44 -> Runnable_IMAP_10ms_sys/134(SDFAve_g_R0_MARK_WIDTH)  "<SDFAve_g_R0_MARK_WIDTH (signal 47)>"
  Bus Selector1/45 -> Runnable_IMAP_10ms_sys/135(SDFAve_g_L1_C0_COEF)  "<SDFAve_g_R0_VIEW_RANGE (signal 48)>"
  Bus Selector1/46 -> Runnable_IMAP_10ms_sys/136(SDFAve_g_L1_C1_COEF)  "<SDFAve_g_L1_C1_COEF (signal 49)>"
  Bus Selector1/47 -> Runnable_IMAP_10ms_sys/137(SDFAve_g_L1_C2_COEF)  "<SDFAve_g_L1_C2_COEF (signal 50)>"
  Bus Selector1/48 -> Runnable_IMAP_10ms_sys/138(SDFAve_g_L1_C3_COEF)  "<SDFAve_g_L1_C3_COEF (signal 51)>"
  Bus Selector1/49 -> Runnable_IMAP_10ms_sys/139(SDFAve_g_L1_VIEW_RANGE)  "<SDFAve_g_L1_VIEW_RANGE (signal 52)>"
  Bus Selector1/50 -> Runnable_IMAP_10ms_sys/140(SDFAve_y_L1_DETECT_QUALITY)  "<SDFAve_y_L1_DETECT_QUALITY (signal 53)>"
  Bus Selector1/51 -> Runnable_IMAP_10ms_sys/141(SDFAve_d_L1_LINE_TYPE)  "<SDFAve_d_L1_LINE_TYPE (signal 54)>"
  Bus Selector1/52 -> Runnable_IMAP_10ms_sys/142(SDFAve_g_L1_MARK_WIDTH)  "<SDFAve_g_L1_MARK_WIDTH (signal 55)>"
  Bus Selector1/53 -> Runnable_IMAP_10ms_sys/143(SDFAve_g_R1_C0_COEF)  "<SDFAve_g_R1_C0_COEF (signal 56)>"
  Bus Selector1/54 -> Runnable_IMAP_10ms_sys/144(SDFAve_g_R1_C1_COEF)  "<SDFAve_g_R1_C1_COEF (signal 57)>"
  Bus Selector1/55 -> Runnable_IMAP_10ms_sys/145(SDFAve_g_R1_C2_COEF)  "<SDFAve_g_R1_C2_COEF (signal 58)>"
  Bus Selector1/56 -> Runnable_IMAP_10ms_sys/146(SDFAve_g_R1_C3_COEF)  "<SDFAve_g_R1_C3_COEF (signal 59)>"
  Bus Selector1/57 -> Runnable_IMAP_10ms_sys/147(SDFAve_g_R1_VIEW_RANGE)  "<SDFAve_g_R1_VIEW_RANGE (signal 60)>"
  Bus Selector1/58 -> Runnable_IMAP_10ms_sys/148(SDFAve_y_R1_DETECT_QUALITY)  "<SDFAve_y_R1_DETECT_QUALITY (signal 61)>"
  Bus Selector1/59 -> Runnable_IMAP_10ms_sys/149(SDFAve_d_R1_LINE_TYPE)  "<SDFAve_d_R1_LINE_TYPE (signal 62)>"
  Bus Selector1/60 -> Runnable_IMAP_10ms_sys/150(SDFAve_g_R1_MARK_WIDTH)  "<SDFAve_g_R1_MARK_WIDTH (signal 63)>"
  Bus Selector1/61 -> Runnable_IMAP_10ms_sys/151(SDFAve_g_L0_C0_BACK_COEF)  "<SDFAve_g_L0_C0_BACK_COEF (signal 64)>"
  Bus Selector1/62 -> Runnable_IMAP_10ms_sys/152(SDFAve_g_L0_C1_BACK_COEF)  "<SDFAve_g_L0_C1_BACK_COEF (signal 65)>"
  Bus Selector1/63 -> Runnable_IMAP_10ms_sys/153(SDFAve_g_L0_C2_BACK_COEF)  "<SDFAve_g_L0_C2_BACK_COEF (signal 66)>"
  Bus Selector1/64 -> Runnable_IMAP_10ms_sys/154(SDFAve_g_L0_C3_BACK_COEF)  "<SDFAve_g_L0_C3_BACK_COEF (signal 67)>"
  Bus Selector1/65 -> Runnable_IMAP_10ms_sys/155(SDFAve_g_L0_BACK_RANGE)  "<SDFAve_g_L0_BACK_RANGE (signal 68)>"
  Bus Selector1/66 -> Runnable_IMAP_10ms_sys/156(SDFAve_g_R0_C0_BACK_COEF)  "<SDFAve_g_R0_C0_BACK_COEF (signal 69)>"
  Bus Selector1/67 -> Runnable_IMAP_10ms_sys/157(SDFAve_g_R0_C1_BACK_COEF)  "<SDFAve_g_R0_C1_BACK_COEF (signal 70)>"
  Bus Selector1/68 -> Runnable_IMAP_10ms_sys/158(SDFAve_g_R0_C2_BACK_COEF)  "<SDFAve_g_L0_C0_BACK_COEF (signal 71)>"
  Bus Selector1/69 -> Runnable_IMAP_10ms_sys/159(SDFAve_g_R0_C3_BACK_COEF)  "<SDFAve_g_R0_C3_BACK_COEF (signal 72)>"
  Bus Selector1/70 -> Runnable_IMAP_10ms_sys/160(SDFAve_g_R0_BACK_RANGE)  "<SDFAve_g_R0_BACK_RANGE (signal 73)>"
  Bus Selector1/71 -> Runnable_IMAP_10ms_sys/161(SDFAve_g_L1_C0_BACK_COEF)  "<SDFAve_g_L1_C0_BACK_COEF (signal 74)>"
  Bus Selector1/72 -> Runnable_IMAP_10ms_sys/162(SDFAve_g_L1_C1_BACK_COEF)  "<SDFAve_g_L1_C1_BACK_COEF (signal 75)>"
  Bus Selector1/73 -> Runnable_IMAP_10ms_sys/163(SDFAve_g_L1_C2_BACK_COEF)  "<SDFAve_g_L1_C2_BACK_COEF (signal 76)>"
  Bus Selector1/74 -> Runnable_IMAP_10ms_sys/164(SDFAve_g_L1_C3_BACK_COEF)  "<SDFAve_g_L1_C3_BACK_COEF (signal 77)>"
  Bus Selector1/75 -> Runnable_IMAP_10ms_sys/165(SDFAve_g_L1_BACK_RANGE)  "<SDFAve_g_L1_BACK_RANGE (signal 78)>"
  Bus Selector1/76 -> Runnable_IMAP_10ms_sys/166(SDFAve_g_R1_C0_BACK_COEF)  "<SDFAve_g_R1_C0_BACK_COEF (signal 79)>"
  Bus Selector1/77 -> Runnable_IMAP_10ms_sys/167(SDFAve_g_R1_C1_BACK_COEF)  "<SDFAve_g_R1_C1_BACK_COEF (signal 80)>"
  Bus Selector1/78 -> Runnable_IMAP_10ms_sys/168(SDFAve_g_R1_C2_BACK_COEF)  "<SDFAve_g_R1_C2_BACK_COEF (signal 81)>"
  Bus Selector1/79 -> Runnable_IMAP_10ms_sys/169(SDFAve_g_R1_C3_BACK_COEF)  "<SDFAve_g_R1_C3_BACK_COEF (signal 82)>"
  Bus Selector1/80 -> Runnable_IMAP_10ms_sys/170(SDFAve_g_R1_BACK_RANGE)  "<SDFAve_g_R1_BACK_RANGE (signal 83)>"
  Data Type  Conversion7/1 -> Runnable_IMAP_10ms_sys/59(SWINve_y_ESC_EPBStaus)  "ESC_EPBStaus"
  BCM_IgnitionSt/1 -> Data Type  Conversion22/1  "BCM_IgnitionSt"
  Data Type  Conversion105/1 -> Runnable_IMAP_10ms_sys/76(SWINve_y_TCU_ATFailure)  "TCU_ATFailure"
  Read CM Dict23/1 -> Data Type  Conversion49/1  "ESC_BrakeOilPress"
  ESC_RLWHeelPulseCounterValidity/1 -> Data Type  Conversion98/1  "ESC_RLWHeelPulseCounterValidity"
  EMS_ACCFunctionIhibition/1 -> Data Type  Conversion21/1  "EMS_ACCFunctionIhibition"
  Data Type  Conversion98/1 -> Runnable_IMAP_10ms_sys/64(SWINve_y_ESC_RLWHeelPulseCounterValidity)  "ESC_RLWHeelPulseCounterValidity"
  Data Type  Conversion112/1 -> Runnable_IMAP_10ms_sys/84(SWINve_y_ESC_VehDrivingDirection)  "ESC_VehDrivingDirection"
  Read CM Dict20/1 -> Gain1/1  "SAS_SteeringAngle"
  Data Type  Conversion115/1 -> Runnable_IMAP_10ms_sys/87(SWINve_y_ESC_VehSpdValidFlag)  "ESC_VehSpdValidFlag"
  Data Type  Conversion45/1 -> Runnable_IMAP_10ms_sys/82(SWINve_y_EPS_TorqueLimitationState)  "EPS_TorqueLimitationState"
  Read CM Dict26/1 -> Subsystem16/1(DM.Gas)  "EMS_ACCResponseStatus"
  Data Type  Conversion106/1 -> Runnable_IMAP_10ms_sys/77(SWINve_y_GW_TCU_DCTClutchStatus)  "GW_TCU_DCTClutchStatus"
  Data Type  Conversion104/1 -> Runnable_IMAP_10ms_sys/75(SWINve_y_TCU_TargetGear)  "TCU_TargetGear"
  Data Type  Conversion50/1 -> Runnable_IMAP_10ms_sys/69(SWINve_y_ESC_Static_slope)  "ESC_Static_Slope"
  Data Type  Conversion42/1 -> Runnable_IMAP_10ms_sys/73(SWINve_y_SAS_CalibratedStatus)  "SAS_CalibratedStatus"
  Data Type  Conversion57/1 -> Runnable_IMAP_10ms_sys/70(SWINve_g_SAS_SteeringAngle)  "SAS_SteeringAngle"
  Data Type  Conversion36/1 -> Runnable_IMAP_10ms_sys/68(SWINve_y_EPS_LKAState)  "EPS_LKAState"
  Data Type  Conversion90/1 -> Runnable_IMAP_10ms_sys/52(SWINve_y_MP5_AEBSwitch)  "MP5_AEBSwitch"
  ACU_PassengerBeltSwitchSig/1 -> Data Type  Conversion15/1  "ACU_PassengerBeltSwitchSig"
  ESC_BrakingEffort/1 -> Data Type  Conversion64/1  "ESC_BrakingEffort"
  EMS_NotControlableMinPowertra/1 -> Data Type  Conversion83/1  "EMS_NotControlableMinPowertra"
  SAS_SASFailureSts/1 -> Data Type  Conversion19/1  "SAS_SASFailureSts"
  Data Type  Conversion47/1 -> Runnable_IMAP_10ms_sys/86(SWINve_g_ESC_VeSpd)  "ESC_VeSpd"
  Data Type Conversion67/1 -> Runnable_IMAP_10ms_sys/78(SWINve_y_TCU_ActialGear)  "TCU_ActialGear"
  Data Type  Conversion54/1 -> Runnable_IMAP_10ms_sys/61(SWINve_d_ESC_FRWHeelPulseCounter)  "ESC_FRWHeelPulseCounter"
  Data Type  Conversion64/1 -> Runnable_IMAP_10ms_sys/10(SWINve_y_ESC_BrakingEffort)  "ESC_BrakingEffort"
  Data Type  Conversion82/1 -> Runnable_IMAP_10ms_sys/25(SWINve_g_EMS_MinPowertrainWheelTorque)  "EMS_MinPowertrainWheelTorque"
  ESC_EPBStaus/1 -> Data Type  Conversion7/1  "ESC_EPBStaus"
  EMS_LowerestGearMaxTorque/1 -> Data Type  Conversion20/1  "EMS_LowerestGearMaxTorque"
  EMS_AccPedalPos/1 -> Gain10/1  "EMS_AccPedalPos"
  Data Type  Conversion89/1 -> Runnable_IMAP_10ms_sys/51(SWINve_y_ESC_BrakeReleasedFailsafe)  "ESC_BrakeReleasedFailsafe"
  Gain7/1 -> Data Type  Conversion95/1  "RearRightWheelSpd"
  Read CM Dict3/1 -> Gain/1  "EMS_BrakePedalSignal"
  TCU_GearEngagement/1 -> Data Type  Conversion109/1  "TCU_GearEngagement"
  Data Type  Conversion60/1 -> Runnable_IMAP_10ms_sys/8(SWINve_y_BCM_HazardLampSt)  "BCM_HazardLampSt"
  Data Type  Conversion91/1 -> Runnable_IMAP_10ms_sys/53(SWINve_y_ESC_MSRinRegulation)  "MSRinRegulation"
  Data Type  Conversion93/1 -> Runnable_IMAP_10ms_sys/55(SWINve_g_ESC_FrontRightWHeelSpd)  "FrontRightWHeelSpd"
  Gain2/1 -> Data Type  Conversion47/1  "ESC_VeSpd"
  Data Type  Conversion86/1 -> Runnable_IMAP_10ms_sys/49(SWINve_y_Mp5_LSSMode)  "Mp5_LSSMode"
  Gain8/1 -> Data Type  Conversion77/1  "EMS_EngSpd"
  GW_SCC_RightSteeringWheelSwitch/1 -> Data Type  Conversion11/1  "SCC_RightSteeringWheelSwitchSig"
  2/1 -> Gain5/1
  Subsystem17/1(TCU_Gear_lever_position) -> Data Type Conversion67/1  "TCU_ActialGear"
  Data Type Conversion9/1 -> Runnable_IMAP_10ms_sys/15(SWINve_g_EMS_AccPedalPositionRaw)  "EMS_AccPedalPositionRaw"
  Data Type  Conversion55/1 -> Runnable_IMAP_10ms_sys/62(SWINve_d_ESC_RLWHeelPulseCounter)  "ESC_RLWHeelPulseCounter"
  Data Type  Conversion96/1 -> Runnable_IMAP_10ms_sys/58(SWINve_g_IC_TotalOdemeter)  "IC_TotalOdemeter"
  Read CM Dict32/1 -> Data Type  Conversion37/1  "EPS_SteeringTorqueValue"
  Data Type  Conversion12/1 -> Runnable_IMAP_10ms_sys/42(SWINve_y_BCM_HighBeamStatus)  "BCM_HighBeamStatus"
  Data Type  Conversion113/1 -> Runnable_IMAP_10ms_sys/85(SWINve_y_ESC_VehicleHoldStatus)  "ESC_VehicleHoldStatus"
  Data Type  Conversion87/1 -> Runnable_IMAP_10ms_sys/50(SWINve_y_Mp5_LSSSwitch)  "Mp5_LSSSwitch"
  Data Type  Conversion73/1 -> Runnable_IMAP_10ms_sys/17(SWINve_d_EMS_RealizedPowertrainWheelTorq)  "EMS_RealizedPowertrainWheelTorq"
  ESC_VehSpdValidFlag/1 -> Data Type  Conversion115/1  "ESC_VehSpdValidFlag"
  GW_TCU_DCTClutchStatus/1 -> Data Type  Conversion106/1  "GW_TCU_DCTClutchStatus"
  Read CM Dict28/1 -> Subsystem17/1(In1)
  ESC_ESCOFF/1 -> Data Type  Conversion295/1  "ESC_ESCOFF"
  Data Type  Conversion101/1 -> Runnable_IMAP_10ms_sys/66(SWINve_y_ESC_ESCAlarmSig)  "ESC_ABSAlarmSig"
  Subsystem15/1(EMS_WhetherACCRequestRealized) -> Data Type Conversion92/1  "EMS_WhetherACCRequestRealized"
  MP5_FCWSensitivity/1 -> Data Type  Conversion14/1  "MP5_FCWSensitivity"
  EMS_EngRunningStatus/1 -> Data Type  Conversion78/1  "EMS_EngRunningStatus"
  Data Type  Conversion63/1 -> Runnable_IMAP_10ms_sys/9(SWINve_y_EMS_BrakePedalSignal)  "EMS_BrakePedalSignal"
  Data Type  Conversion77/1 -> Runnable_IMAP_10ms_sys/20(SWINve_g_EMS_EngSpd)  "EMS_EngSpd"
  Data Type  Conversion76/1 -> Runnable_IMAP_10ms_sys/19(SWINve_g_EMS_DriverTorque)  "EMS_DriverTorque"
  Data Type  Conversion75/1 -> Runnable_IMAP_10ms_sys/18(SWINve_g_EMS_AccPedalPos)  "EMS_AccPedalPos"
  Data Type  Conversion51/1 -> Runnable_IMAP_10ms_sys/11(SWINve_y_ESC_DynamicSlope)  "ESC_DynamicSlope"
  Data Type Conversion92/1 -> Runnable_IMAP_10ms_sys/13(SWINve_y_EMS_WhetherACCRequestRealized)  "EMS_WhetherACCRequestRealized/EMS_ACC_Effecitive_EMS"
  Data Type  Conversion294/1 -> Runnable_IMAP_10ms_sys/4(SWINve_y_ESC_TCSCtlActive)  "ESC_TCSCtlActive"
  Data Type  Conversion48/1 -> Runnable_IMAP_10ms_sys/2(SWINve_g_ESC_LongitudinalAcceleration)  "ESC_LongitudinalAcceleration"
  Data Type  Conversion56/1 -> Runnable_IMAP_10ms_sys/63(SWINve_d_ESC_RRWHeelPulseCounter)  "ESC_RRWHeelPulseCounter"
  ESC_ABSWorkLable/1 -> Data Type  Conversion297/1  "ESC_ABSWorkLable"
  Subsystem18/1(EMS_WhlTrq_max) -> Data Type  Conversion80/1  "EMS_MaxPowertrainWheelTorque"
  Data Type  Conversion26/1 -> Runnable_IMAP_10ms_sys/27(SWINve_y_ESC_ESCWorkStatus)  "ESC_ESCWorkStatus"
  Data Type  Conversion81/1 -> Runnable_IMAP_10ms_sys/24(SWINve_g_EMS_NotControlableMaxPowertra)  "EMS_NotControlableMaxPowertra"
  Data Type  Conversion80/1 -> Runnable_IMAP_10ms_sys/23(SWINve_g_EMS_MaxPowertrainWheelTorque)  "EMS_MaxPowertrainWheelTorque"
  EMS_ACCcontrolTorqueAvailable/1 -> Data Type  Conversion71/1  "EMS_ACCcontrolTorqueAvailable"
  Data Type  Conversion46/1 -> Runnable_IMAP_10ms_sys/48(SWINve_g_ESC_LateralAccelaration)  "ESC_LateralAccelaration"
  Data Type  Conversion99/1 -> Runnable_IMAP_10ms_sys/65(SWINve_y_ESC_RRWHeelPulseCounterValidity)  "ESC_RRWHeelPulseCounterValidity"
  ESC_RLWHeelPulseCounter/1 -> Data Type  Conversion55/1  "ESC_RLWHeelPulseCounter"
  Data Type  Conversion19/1 -> Runnable_IMAP_10ms_sys/47(SWINve_y_SAS_SASFailureSts)  "SAS_SASFailureSts"
  Data Type  Conversion16/1 -> Runnable_IMAP_10ms_sys/46(SWINve_y_ACU_DriverBeltSwitchSig)  "ACU_DriverBeltSwitchSig"
  Data Type  Conversion14/1 -> Runnable_IMAP_10ms_sys/44(SWINve_y_MP5_FCWSensitivity)  "MP5_FCWSensitivity"
  Data Type  Conversion11/1 -> Runnable_IMAP_10ms_sys/38(SWINve_y_SCC_RightSteeringWheelSwitchSig)  "SCC_RightSteeringWheelSwitchSig"
  Data Type  Conversion9/1 -> Runnable_IMAP_10ms_sys/36(SWINve_y_Mp5_TSRSwitch)  "Mp5_TSRSwitch"
  Saturation/1 -> Data Type  Conversion58/1
  Data Type  Conversion8/1 -> Runnable_IMAP_10ms_sys/35(SWINve_y_Mp5_ISASwitch)  "Mp5_ISASwitch"
  Read CM Dict14/1 -> Gain2/1
  Data Type  Conversion27/1 -> Runnable_IMAP_10ms_sys/34(SWINve_g_EMS_HighestGearMinTorque)  "EMS_HighestGearMinTorque"
  Data Type Conversion4/1 -> Runnable_IMAP_10ms_sys/32(SWINve_y_EMS_ACCResponseStatus)  "EMS_ACCResponseStatus"
  Data Type  Conversion24/1 -> Runnable_IMAP_10ms_sys/29(SWINve_y_ESC_FRWHeelPulseCounterValidity)  "ESC_FRWHeelPulseCounterValidity"
  Data Type  Conversion25/1 -> Runnable_IMAP_10ms_sys/28(SWINve_y_ESC_FLWHeelPulseCounterValidity)  "ESC_FLWHeelPulseCounterValidity"
  Data Type  Conversion108/1 -> Runnable_IMAP_10ms_sys/80(SWINve_y_TCU_SelectedATMode)  "TCU_SelectedATMode"
  Data Type  Conversion290/1 -> Runnable_IMAP_10ms_sys/7(SWINve_y_BCM_FrontWiperWorkSt)  "BCM_FrontWiperWorkSt"
  Data Type  Conversion41/1 -> Runnable_IMAP_10ms_sys/60(SWINve_d_ESC_FLWHeelPulseCounter)  "ESC_FLWHeelPulseCounter"
  Saturation1/1 -> Data Type  Conversion57/1
  Gain/1 -> Subsystem24/1(Inport)
  Data Type  Conversion13/1 -> Runnable_IMAP_10ms_sys/43(SWINve_y_MP5_FCWSwitch)  "MP5_FCWSwitch"
  3/1 -> Gain6/1
  ESC_VehicleHoldStatus/1 -> Data Type  Conversion113/1  "ESC_VehicleHoldStatus"
  ESC_Static_slope/1 -> Gain12/1  "ESC_Static_Slope"
  ESC_VehDrivingDirection/1 -> Data Type  Conversion112/1  "ESC_VehDrivingDirection"
  Subsystem19/1(TCU_AGB_Target_position) -> Data Type  Conversion104/1  "TCU_TargetGear"
  ESC_DynamicSlope/1 -> Gain11/1  "ESC_DynamicSlope"
  ESC_BrakeReleasedFailsafe/1 -> Data Type  Conversion89/1  "ESC_BrakeReleasedFailsafe"
  ACCEL_LONGI_CALIB1/1 -> Data Type  Conversion48/1  "ACCEL_LONGI_CALIB"
  ESC_RRWHeelPulseCounter/1 -> Data Type  Conversion56/1  "ESC_RRWHeelPulseCounter"
  MSRinRegulation/1 -> Data Type  Conversion91/1  "MSRinRegulation"
  TCU_SelectedATMode/1 -> Data Type  Conversion108/1  "TCU_SelectedATMode"
  BCM_HighBeamStatus/1 -> Data Type  Conversion12/1  "BCM_HighBeamStatus"
  1/1 -> Gain4/1
  Gain6/1 -> Data Type  Conversion94/1  "ESC_RearLeftWheelSpd"
  Read CM Dict19/1 -> Gain3/1  "SAS_SteeringRotSpd"
  EMS_ACCcontrolGearAvailable/1 -> Data Type  Conversion79/1  "EMS_ACCcontrolGearAvailable"
  Mp5_TSRSwitch/1 -> Data Type  Conversion9/1  "Mp5_TSRSwitch"
  Data Type  Conversion79/1 -> Runnable_IMAP_10ms_sys/22(SWINve_y_EMS_ACCcontrolGearAvailable)  "EMS_ACCcontrolGearAvailable"
  Read CM Dict11/1 -> Subsystem21/1(In1)  "EMS_RealizedPowertrainWheelTorq"
  Gain5/1 -> Data Type  Conversion93/1  "FrontRightWHeelSpd"
  Subsystem21/1(TCU_AGB_position) -> Data Type  Conversion73/1  "EMS_RealizedPowertrainWheelTorq"
  Constant10/1 -> Switch/1
  Read CM Dict6/1 -> Switch/2
  Read CM Dict5/1 -> Gain9/1
  TCU_ATFailure/1 -> Data Type  Conversion105/1  "TCU_ATFailure"
  ESC_DynamicSlopeAccuracy/1 -> Data Type  Conversion52/1  "ESC_DynamicSlopeAccuracy"
  Subsystem16/1(EMS_ACCResponseStatus) -> Data Type Conversion4/1  "EMS_ACCResponseStatus"
  Constant1/1 -> Switch/3
  EPS_TorqueLimitationState/1 -> Data Type  Conversion45/1  "EPS_TorqueLimitationState"
  Read CM Dict16/1 -> Gain8/1  "EMS_EngSpd"
  ESC_FLWHeelPulseCounterValidity/1 -> Data Type  Conversion25/1  "ESC_FLWHeelPulseCounterValidity"
  Read CM Dict7/1 -> Data Type  Conversion60/1  "BCM_HazardLampSt"
  Gain4/1 -> Data Type  Conversion92/1  "ESC_FrontLeftWHeelSpd"
  Read CM Dict22/1 -> Data Type  Conversion8/1  "Mp5_ISASwitch"
  ESC_FRWHeelPulseCounter/1 -> Data Type  Conversion54/1  "ESC_FRWHeelPulseCounter"
  ACU_DriverBeltSwitchSig/1 -> Data Type  Conversion16/1  "ACU_DriverBeltSwitchSig"
  ESC_FLWHeelPulseCounter/1 -> Data Type  Conversion41/1  "ESC_FLWHeelPulseCounter"
  Gain3/1 -> Saturation/1
  ESC_TCSCtlActive/1 -> Data Type  Conversion294/1  "ESC_TCSCtlActive"
  Data Type  Conversion44/1 -> Runnable_IMAP_10ms_sys/74(SWINve_y_SAS_TrimmingStatus)  "SAS_TrimmingStatus"
  Read CM Dict9/1 -> Subsystem18/1(In1)
  Data Type  Conversion94/1 -> Runnable_IMAP_10ms_sys/56(SWINve_g_ESC_RearLeftWheelSpd)  "ESC_RearLeftWheelSpd"
  Front_right_pulse_malfunction/1 -> Data Type  Conversion24/1  "ESC_FRWHeelPulseCounterValidity"
  Data Type  Conversion72/1 -> Runnable_IMAP_10ms_sys/16(SWINve_g_EMS_EngActualFlwTorque)  "EMS_EngActualFlwTorque"
  Compare To Constant2/1 -> Data Type  Conversion103/1  "EPS_SteeringHoldState"
  Subsystem24/1(Brake_secondary_contact) -> Data Type  Conversion63/1  "EMS_BrakePedalSignal"
  EMS_HighestGearMinTorque/1 -> Data Type  Conversion27/1  "EMS_HighestGearMinTorque"
  ESC_LateralAccelaration/1 -> Data Type  Conversion46/1  "ESC_LateralAccelaration"
  Data Type  Conversion297/1 -> Runnable_IMAP_10ms_sys/1(SWINve_y_ESC_ABSWorkLable)  "ESC_ABSWorkLable"
  4/1 -> Gain7/1
  ESC_RRWHeelPulseCounterValidity/1 -> Data Type  Conversion99/1  "ESC_RRWHeelPulseCounterValidity"
  SAS_CalibratedStatus/1 -> Data Type  Conversion42/1  "SAS_CalibratedStatus"
  Data Type  Conversion293/1 -> Runnable_IMAP_10ms_sys/5(SWINve_y_BCM_BrakeLampStaus)  "BCM_BrakeLampStatus"
  Data Type  Conversion78/1 -> Runnable_IMAP_10ms_sys/21(SWINve_y_EMS_EngRunningStatus)  "EMS_EngRunningStatus"
  Read CM Dict4/1 -> Data Type  Conversion10/1  "SCC_LeftSteeringWheelSwitchSig"
  Data Type  Conversion52/1 -> Runnable_IMAP_10ms_sys/12(SWINve_y_ESC_DynamicSlopeAccuracy)  "ESC_DynamicSlopeAccuracy"
  Data Type  Conversion71/1 -> Runnable_IMAP_10ms_sys/14(SWINve_y_EMS_ACCcontrolTorqueAvailable)  "EMS_ACCcontrolTorqueAvailable"
  Data Type  Conversion58/1 -> Runnable_IMAP_10ms_sys/71(SWINve_g_SAS_SteeringRotSpd)  "SAS_SteeringRotSpd"
  Read CM Dict10/1 -> Data Type  Conversion72/1  "EMS_EngActualFlwTorque"
  IC_TotalOdemeter/1 -> Data Type  Conversion96/1  "IC_TotalOdemeter"
  BCM_CHMSLStatus/1 -> Data Type  Conversion292/1  "BCM_CHMSLStatus"
  Data Type  Conversion110/1 -> Runnable_IMAP_10ms_sys/83(SWINve_y_ESC_VehicleStandstill)  "ESC_VehicleStandstill"
  Read CM Dict24/1 -> ACCEL_LONGI_CALIB1/1
  Data Type  Conversion292/1 -> Runnable_IMAP_10ms_sys/6(SWINve_y_BCM_CHMSLStaus)  "BCM_CHMSLStatus"
  Data Type  Conversion21/1 -> Runnable_IMAP_10ms_sys/31(SWINve_y_EMS_ACCFunctionIhibition)  "EMS_ACCFunctionIhibition"
  Data Type  Conversion103/1 -> Runnable_IMAP_10ms_sys/67(SWINve_y_EPS_SteeringHoldState)  "EPS_SteeringHoldState"
  Data Type  Conversion15/1 -> Runnable_IMAP_10ms_sys/45(SWINve_y_ACU_PassengerBeltSwitchSig)  "ACU_PassengerBeltSwitchSig"
  Data Type  Conversion20/1 -> Runnable_IMAP_10ms_sys/33(SWINve_g_EMS_LowerestGearMaxTorque)  "EMS_LowerestGearMaxTorque"
  Data Type  Conversion37/1 -> Runnable_IMAP_10ms_sys/72(SWINve_g_EPS_SteeringTorqueValue)  "EPS_SteeringTorqueValue"
  BCM_FrontWiperWorkSt/1 -> Data Type  Conversion290/1  "BCM_FrontWiperWorkSt"
  SAS_TrimmingStatus/1 -> Data Type  Conversion44/1  "SAS_TrimmingStatus"
  Data Type  Conversion295/1 -> Runnable_IMAP_10ms_sys/3(SWINve_y_ESC_ESCOFF)  "ESC_ESCOFF"
  Data Type  Conversion83/1 -> Runnable_IMAP_10ms_sys/26(SWINve_g_EMS_NotControlableMinPowertra)  "EMS_NotControlableMinPowertra"
  Switch/1 -> Data Type  Conversion110/1  "ESC_VehicleStandstill"
  BCM_BrakeLampStatus/1 -> Data Type  Conversion293/1  "BCM_BrakeLampStatus"
  Data Type  Conversion109/1 -> Runnable_IMAP_10ms_sys/79(SWINve_y_TCU_GearEngagement)  "TCU_GearEngagement"
  Data Type  Conversion22/1 -> Runnable_IMAP_10ms_sys/30(SWINve_y_BCM_IgnitionSt)  "BCM_IgnitionSt"
  Read CM Dict17/1 -> Subsystem19/1(In1)
  ESC_ESCWorkStatus/1 -> Data Type  Conversion26/1  "ESC_ESCWorkStatus"
  Gain1/1 -> Saturation1/1
  Data Type  Conversion92/1 -> Runnable_IMAP_10ms_sys/54(SWINve_g_ESC_FrontLeftWHeelSpd)  "ESC_FrontLeftWHeelSpd"
  EMS_DriverTorque/1 -> Data Type  Conversion76/1  "EMS_DriverTorque"
  EMS_NotControlableMaxPowertra/1 -> Data Type  Conversion81/1  "EMS_NotControlableMaxPowertra"
  ESC_ABSAlarmSig/1 -> Data Type  Conversion101/1  "ESC_ABSAlarmSig"
  Subsystem18/2(EMS_WhlTrq_min) -> Data Type  Conversion82/1  "EMS_MinPowertrainWheelTorque"
  Read CM Dict1/1 -> Data Type  Conversion36/1  "EPS_LKAState"
  Data Type  Conversion95/1 -> Runnable_IMAP_10ms_sys/57(SWINve_g_ESC_RearRightWheelSpd)  "RearRightWheelSpd"
  Data Type  Conversion10/1 -> Runnable_IMAP_10ms_sys/37(SWINve_y_SCC_LeftSteeringWheelSwitchSig)  "SCC_LeftSteeringWheelSwitchSig"
  Data Type  Conversion49/1 -> Runnable_IMAP_10ms_sys/81(SWINve_g_ESC_BrakeOilPress)  "ESC_BrakeOilPress"
  BusCreator/1 -> IMAP_Output/1
  Subsystem208/1(obj_Dx) -> Data Type Conversion35/1
  Subsystem203/1(obj_abs_Ax) -> Data Type Conversion24/1
  Subsystem160/1(obj_Rel_Vx) -> Data Type Conversion224/1
  Subsystem210/1(obj_Dy) -> Data Type Conversion37/1
  Subsystem204/1(obj_abs_Ay) -> Data Type Conversion33/1
  Subsystem192/1(obj_Rel_Vy) -> Data Type Conversion246/1
  Data Type Conversion24/1 -> Runnable_IMAP_10ms_sys/299(SDFAva_g_ORI_Obj_AbsAx)  "IFC_obj_abs_Ax"
  Data Type Conversion33/1 -> Runnable_IMAP_10ms_sys/300(SDFAva_g_ORI_Obj_AbsAy)  "IFC_obj_abs_Ay"
  Data Type Conversion224/1 -> Runnable_IMAP_10ms_sys/301(SDFAva_g_ORI_Obj_RelVel)  "IFC_obj_Rel_Vx"
  Data Type Conversion246/1 -> Runnable_IMAP_10ms_sys/302(SDFAva_g_ORI_Obj_RelVely)  "IFC_obj_Rel_Vy"
  Data Type Conversion35/1 -> Runnable_IMAP_10ms_sys/303(SDFAva_g_ORI_Obj_LongDis)  "IFC_obj_Dx"
  Data Type Conversion37/1 -> Runnable_IMAP_10ms_sys/304(SDFAva_g_ORI_Obj_LateralDis)  "IFC_obj_Dy"
  Data Type Conversion216/1 -> Runnable_IMAP_10ms_sys/315(SDFAve_d_ORI_L1_Type)  "IFC_Line03_Type"
  Data Type Conversion26/1 -> Runnable_IMAP_10ms_sys/316(SDFAve_g_ORI_L1_VR)  "VR_L1"
  Data Type Conversion223/1 -> Runnable_IMAP_10ms_sys/317(SDFAve_g_ORI_R0_C3)  "IFC_Line02_CurvChange"
  Data Type Conversion225/1 -> Runnable_IMAP_10ms_sys/318(SDFAve_g_ORI_R0_C2)  "IFC_Line02_Curv"
  Data Type Conversion226/1 -> Runnable_IMAP_10ms_sys/319(SDFAve_g_ORI_R0_C1)  "IFC_Line02_HeadingAngle"
  Data Type Conversion227/1 -> Runnable_IMAP_10ms_sys/320(SDFAve_g_ORI_R0_C0)  "IFC_Line02_Dy"
  Data Type Conversion230/1 -> Runnable_IMAP_10ms_sys/321(SDFAve_d_ORI_R0_LT)  "IFC_Line03_Type"
  Data Type Conversion25/1 -> Runnable_IMAP_10ms_sys/322(SDFAve_g_ORI_R0_VR)  "R0_VR"
  Data Type Conversion238/1 -> Runnable_IMAP_10ms_sys/323(SDFAve_g_ORI_R1_C3)  "IFC_Line04_CurvChange"
  Data Type Conversion239/1 -> Runnable_IMAP_10ms_sys/324(SDFAve_g_ORI_R1_C2)  "IFC_Line04_Curv"
  Data Type Conversion240/1 -> Runnable_IMAP_10ms_sys/325(SDFAve_g_ORI_R1_C1)  "IFC_Line04_HeadingAngle"
  Data Type Conversion241/1 -> Runnable_IMAP_10ms_sys/326(SDFAve_g_ORI_R1_C0)  "IFC_Line04_Dy"
  Data Type Conversion244/1 -> Runnable_IMAP_10ms_sys/327(SDFAve_d_ORI_R1_LT)  "IFC_Line04_Type"
  Data Type Conversion23/1 -> Runnable_IMAP_10ms_sys/328(SDFAve_g_ORI_R1_VR)  "R1_VR"
  [EPS_LKA_State_lka] -> Data Type Conversion/1
  Data Type Conversion38/1 -> Runnable_IMAP_10ms_sys/237(SWINve_y_MP5_ESASwitch)  "MP5_ESASwitch"
  Read CM Dict2/1 -> Data Type Conversion1/1
  Data Type Conversion2/1 -> Runnable_IMAP_10ms_sys/247(SWINve_y_PEPS_DoorLockReq)
  Read CM Dict8/1 -> Data Type Conversion2/1
  Read CM Dict12/1 -> Data Type Conversion3/1
  Constant2/1 -> Data Type  Conversion3/1
  ESC_LongitudinalAccelervalidity/1 -> Data Type  Conversion4/1
  Data Type  Conversion5/1 -> Runnable_IMAP_10ms_sys/261(SWINve_y_EPS_WarmingLampSt)  "EPS_WarmingLampSt"
  EPS_WarmingLampSt/1 -> Data Type  Conversion5/1
  Data Type Conversion5/1 -> Write CM Dict1/1
  Data Type Conversion6/1 -> Write CM Dict/1
  Data Type Conversion10/1 -> Data Type  Conversion87/1  "Mp5_LSSSwitch"
  Data Type Conversion8/1 -> Data Type  Conversion90/1  "MP5_AEBSwitch"
  Data Type Conversion11/1 -> Data Type  Conversion86/1  "Mp5_LSSMode"
  Read CM Dict27/1 -> Data Type Conversion8/1  "MP5_AEBSwitch"
  Read CM Dict29/1 -> Data Type Conversion10/1  "Mp5_LSSSwitch"
  Data Type Conversion7/1 -> Data Type  Conversion13/1  "MP5_FCWSwitch"
  Read CM Dict30/1 -> Data Type Conversion11/1  "Mp5_LSSMode"
  Read CM Dict31/1 -> Data Type Conversion7/1  "MP5_FCWSwitch"
  Read CM Dict36/1 -> Compare To Constant2/1
  Data Type  Conversion3/1 -> Runnable_IMAP_10ms_sys/214(SWINve_y_BCM_FrontWiperSwitchSt)  "BCM_FrontWiperSwitchSt"
  Data Type Conversion1/1 -> Runnable_IMAP_10ms_sys/238(SWINve_y_Mp5_ELKSwitch)  "Mp5_ELKSwitch"
  Data Type Conversion3/1 -> Runnable_IMAP_10ms_sys/248(SWINve_y_BCM_DoorLockSt)
  Data Type Conversion42/1 -> Runnable_IMAP_10ms_sys/245(SWINve_y_MP5_JA_Alert_Switch)  "MP5_JA_Alert_Switch"
  Data Type Conversion31/1 -> Runnable_IMAP_10ms_sys/279(SWINve_y_ESC_ACCActive)  "ESC_ACCActive"
  Data Type  Conversion133/1 -> Runnable_IMAP_10ms_sys/274(SWINve_y_ESC_RLWHeelSpdFaultSignal)  "ESC_RLWHeelSpdFaultSignal"
  Data Type  Conversion134/1 -> Runnable_IMAP_10ms_sys/275(SWINve_y_ESC_RRWHeelSpdFaultSignal)  "ESC_RRWHeelSpdFaultSignal"
  ESC_ABSAlarmSig1/1 -> Data Type  Conversion6/1  "ESC_ABSAlarmSig"
  Data Type Conversion12/1 -> Manual Switch2/1
  Read CM Dict25/1 -> Data Type Conversion12/1
  Data Type  Conversion2/1 -> Runnable_IMAP_10ms_sys/213(SWINve_y_BCM_RightTurnSwitchSt)
  Data Type  Conversion1/1 -> Runnable_IMAP_10ms_sys/212(SWINve_y_BCM_LeftTurnSwitchSt)
  Read CM Dict15/1 -> Data Type  Conversion2/1  "BCM_RightTurnSwicthSt"
  Read CM Dict13/1 -> Data Type  Conversion1/1  "BCM_LeftTurnSwitchSt"
  Read CM Dict85/1 -> Data Type  Conversion159/1
  Data Type  Conversion159/1 -> Runnable_IMAP_10ms_sys/221(SWINve_y_MP5_AutoPilotSwitch)  "MP5_AutoPilotSwitch"
  Constant23/1 -> Runnable_IMAP_10ms_sys/211(SWINve_y_TCU_TCUAvailable)  "TCU_TCUAvailable"
  Runnable_IMAP_10ms_sys/1(IMAPve_d_LKA_Main_Switch) -> BusCreator/1  "IMAPve_d_LKA_Main_Switch"
  Runnable_IMAP_10ms_sys/2(IMAPve_d_LKA_Mode) -> BusCreator/2  "IMAPve_d_LKA_Mode"
  Runnable_IMAP_10ms_sys/3(IMAPve_d_AEB_Switch) -> BusCreator/3  "IMAPve_d_AEB_Switch"
  Runnable_IMAP_10ms_sys/4(IMAPve_d_FCW_Switch) -> BusCreator/4  "IMAPve_d_FCW_Switch"
  Runnable_IMAP_10ms_sys/5(IMAPve_d_FCW_Sensitivity) -> BusCreator/5  "IMAPve_d_FCW_Sensitivity"
  Runnable_IMAP_10ms_sys/6(IMAPve_d_ISA_Switch) -> BusCreator/6  "IMAPve_d_ISA_Switch"
  Runnable_IMAP_10ms_sys/7(IMAPve_d_TSR_Switch) -> BusCreator/7  "IMAPve_d_TSR_Switch"
  Runnable_IMAP_10ms_sys/8(IMAPve_d_ISA_ISLC_Mode) -> BusCreator/8  "IMAPve_d_ISA_ISLC_Mode"
  Runnable_IMAP_10ms_sys/9(IMAPve_d_LDW_Warn_Mode) -> BusCreator/9  "IMAPve_d_LDW_Warn_Mode"
  Runnable_IMAP_10ms_sys/10(IMAPve_d_Speed_Limit) -> BusCreator/10  "IMAPve_d_Speed_Limit"
  Runnable_IMAP_10ms_sys/11(IMAPve_d_ALC_TLC_Mode) -> BusCreator/11  "IMAPve_d_ALC_TLC_Mode"
  Runnable_IMAP_10ms_sys/12(IMAPve_d_ESA_Switch) -> BusCreator/12  "IMAPve_d_ESA_Switch"
  Runnable_IMAP_10ms_sys/13(IMAPve_d_ELK_Switch) -> BusCreator/13  "IMAPve_d_ELK_Switch"
  Runnable_IMAP_10ms_sys/14(IMAPve_d_PEPS_RKE_Command) -> BusCreator/14  "IMAPve_d_PEPS_RKE_Command"
  Runnable_IMAP_10ms_sys/15(IMAPve_d_BSD_LCW_Switch) -> BusCreator/15  "IMAPve_d_BSD_LCW_Switch"
  Runnable_IMAP_10ms_sys/16(IMAPve_d_FCTA_Switch) -> BusCreator/16  "IMAPve_d_FCTA_Switch"
  Runnable_IMAP_10ms_sys/17(IMAPve_d_RCTA_Swtich) -> BusCreator/17  "IMAPve_d_RCTA_Swtich"
  Runnable_IMAP_10ms_sys/18(IMAPve_d_DOW_Switch) -> BusCreator/18  "IMAPve_d_DOW_Switch"
  Runnable_IMAP_10ms_sys/19(IMAPve_d_JA_Brake_Switch) -> BusCreator/19  "IMAPve_d_JA_Brake_Switch"
  Runnable_IMAP_10ms_sys/20(IMAPve_d_JA_Alert_Switch) -> BusCreator/20  "IMAPve_d_JA_Alert_Switch"
  Data Type Conversion/1 -> BusCreator/21  "IMAPve_d_EPS_LKA_State"
  Runnable_IMAP_10ms_sys/22(IMAPve_g_EPS_SW_Trq) -> BusCreator/22  "IMAPve_g_EPS_SW_Trq"
  Runnable_IMAP_10ms_sys/23(IMAPve_d_EPS_Trq_State) -> BusCreator/23  "IMAPve_d_EPS_Trq_State"
  Runnable_IMAP_10ms_sys/24(IMAPve_d_SAS_Clb_State) -> BusCreator/24  "IMAPve_d_SAS_Clb_State"
  Runnable_IMAP_10ms_sys/25(IMAPve_d_SAS_Trim_State) -> BusCreator/25  "IMAPve_d_SAS_Trim_State"
  Runnable_IMAP_10ms_sys/26(IMAPve_d_EPS_TrqLim_State) -> BusCreator/26  "IMAPve_d_EPS_TrqLim_State"
  Runnable_IMAP_10ms_sys/27(IMAPve_g_EPS_LKA_Current) -> BusCreator/27  "IMAPve_g_EPS_LKA_Current"
  Runnable_IMAP_10ms_sys/28(IMAPve_g_ESC_LatAcc) -> BusCreator/28  "IMAPve_g_ESC_LatAcc"
  Runnable_IMAP_10ms_sys/29(IMAPve_d_ESC_LatAcc_Valid) -> BusCreator/29  "IMAPve_d_ESC_LatAcc_Valid"
  Runnable_IMAP_10ms_sys/30(IMAPve_g_ESC_YawRate) -> BusCreator/30  "IMAPve_g_ESC_YawRate"
  Runnable_IMAP_10ms_sys/31(IMAPve_d_ESC_YawRate_Valid) -> BusCreator/31  "IMAPve_d_ESC_YawRate_Valid"
  Runnable_IMAP_10ms_sys/32(IMAPve_g_ESC_UnYawRate) -> BusCreator/32  "IMAPve_g_ESC_UnYawRate"
  Runnable_IMAP_10ms_sys/33(IMAPve_g_ESC_VehSpd) -> BusCreator/33  "IMAPve_g_ESC_VehSpd"
  Runnable_IMAP_10ms_sys/34(IMAPve_g_ESC_LonAcc) -> BusCreator/34  "IMAPve_g_ESC_LonAcc"
  Runnable_IMAP_10ms_sys/35(IMAPve_d_ESC_LonAcc_Valid) -> BusCreator/35  "IMAPve_d_ESC_LonAcc_Valid"
  Runnable_IMAP_10ms_sys/36(IMAPve_g_ESC_Brake_Press) -> BusCreator/36  "IMAPve_g_ESC_Brake_Press"
  Runnable_IMAP_10ms_sys/37(IMAPve_g_ESC_Static_Slope) -> BusCreator/37  "IMAPve_g_ESC_Static_Slope"
  Runnable_IMAP_10ms_sys/38(IMAPve_g_ESC_DySlope_Accuracy) -> BusCreator/38  "IMAPve_g_ESC_DySlope_Accuracy"
  Runnable_IMAP_10ms_sys/39(IMAPve_g_ESC_DySlope) -> BusCreator/39  "IMAPve_g_ESC_DySlope"
  Runnable_IMAP_10ms_sys/40(IMAPve_g_SW_Angle) -> BusCreator/40  "IMAPve_g_SW_Angle"
  Runnable_IMAP_10ms_sys/41(IMAPve_g_SW_Angle_Speed) -> BusCreator/41  "IMAPve_g_SW_Angle_Speed"
  Runnable_IMAP_10ms_sys/42(IMAPve_d_BCM_HazardLamp) -> BusCreator/42  "IMAPve_d_BCM_HazardLamp"
  Runnable_IMAP_10ms_sys/43(IMAPve_d_BCM_Left_Light) -> BusCreator/43  "IMAPve_d_BCM_Left_Light"
  Runnable_IMAP_10ms_sys/44(IMAPve_d_BCM_Right_Light) -> BusCreator/44  "IMAPve_d_BCM_Right_Light"
  Runnable_IMAP_10ms_sys/45(IMAPve_d_ESC_BrakeLamp_Req) -> BusCreator/45  "IMAPve_d_ESC_BrakeLamp_Req"
  Runnable_IMAP_10ms_sys/46(IMAPve_d_BCM_Opening_State) -> BusCreator/46  "IMAPve_d_BCM_Opening_State"
  Runnable_IMAP_10ms_sys/47(IMAPve_d_BCM_Trunk_State) -> BusCreator/47  "IMAPve_d_BCM_Trunk_State"
  Runnable_IMAP_10ms_sys/48(IMAPve_d_BCM_LF_Door_State) -> BusCreator/48  "IMAPve_d_BCM_LF_Door_State"
  Runnable_IMAP_10ms_sys/49(IMAPve_d_BCM_RF_Door_State) -> BusCreator/49  "IMAPve_d_BCM_RF_Door_State"
  Runnable_IMAP_10ms_sys/50(IMAPve_d_BCM_RR_Door_State) -> BusCreator/50  "IMAPve_d_BCM_RR_Door_State"
  Runnable_IMAP_10ms_sys/51(IMAPve_d_BCM_LR_Door_State) -> BusCreator/51  "IMAPve_d_BCM_LR_Door_State"
  Runnable_IMAP_10ms_sys/52(IMAPve_d_SCC_Left_SwitchSig) -> BusCreator/52  "IMAPve_d_SCC_Left_SwitchSig"
  Runnable_IMAP_10ms_sys/53(IMAPve_d_SCC_Right_SwitchSig) -> BusCreator/53  "IMAPve_d_SCC_Right_SwitchSig"
  Runnable_IMAP_10ms_sys/54(IMAPve_d_BCM_HazardLamp_Switch) -> BusCreator/54  "IMAPve_d_BCM_HazardLamp_Switch"
  Runnable_IMAP_10ms_sys/55(IMAPve_d_PEPS_Door_Lock_Req) -> BusCreator/55  "IMAPve_d_PEPS_Door_Lock_Req"
  Runnable_IMAP_10ms_sys/56(IMAPve_d_BCM_Door_Lock_State) -> BusCreator/56  "IMAPve_d_BCM_Door_Lock_State"
  Runnable_IMAP_10ms_sys/57(IMAPve_d_EMS_ACC_Status) -> BusCreator/57  "IMAPve_d_EMS_ACC_Status"
  Runnable_IMAP_10ms_sys/58(IMAPve_g_EMS_Pot_WhlT_Max) -> BusCreator/58  "IMAPve_g_EMS_Pot_WhlT_Max"
  Runnable_IMAP_10ms_sys/59(IMAPve_g_EMS_Pot_WhlT_Min) -> BusCreator/59  "IMAPve_g_EMS_Pot_WhlT_Min"
  Runnable_IMAP_10ms_sys/60(IMAPve_g_EMS_RealPedal) -> BusCreator/60  "IMAPve_g_EMS_RealPedal"
  Runnable_IMAP_10ms_sys/61(IMAPve_g_EMS_MaxTWhl) -> BusCreator/61  "IMAPve_g_EMS_MaxTWhl"
  Runnable_IMAP_10ms_sys/62(IMAPve_g_EMS_MaxTWhl_Offset) -> BusCreator/62  "IMAPve_g_EMS_MaxTWhl_Offset"
  Runnable_IMAP_10ms_sys/63(IMAPve_g_EMS_MinTWhl) -> BusCreator/63  "IMAPve_g_EMS_MinTWhl"
  Runnable_IMAP_10ms_sys/64(IMAPve_g_EMS_MinTWhl_Offset) -> BusCreator/64  "IMAPve_g_EMS_MinTWhl_Offset"
  Runnable_IMAP_10ms_sys/65(IMAPve_g_EMS_Actual_FlwT) -> BusCreator/65  "IMAPve_g_EMS_Actual_FlwT"
  Runnable_IMAP_10ms_sys/66(IMAPve_g_EMS_Actual_IndT) -> BusCreator/66  "IMAPve_g_EMS_Actual_IndT"
  Runnable_IMAP_10ms_sys/67(IMAPve_g_EMS_Realize_TWhl) -> BusCreator/67  "IMAPve_g_EMS_Realize_TWhl"
  Runnable_IMAP_10ms_sys/68(IMAPve_g_EMS_ACC_VirtualPedal) -> BusCreator/68  "IMAPve_g_EMS_ACC_VirtualPedal"
  Runnable_IMAP_10ms_sys/69(IMAPve_d_EMS_AccPedal_Fault) -> BusCreator/69  "IMAPve_d_EMS_AccPedal_Fault"
  Runnable_IMAP_10ms_sys/70(IMAPve_g_EMS_Driver_Torque) -> BusCreator/70  "IMAPve_g_EMS_Driver_Torque"
  Runnable_IMAP_10ms_sys/71(IMAPve_d_ESC_Brake_Effort) -> BusCreator/71  "IMAPve_d_ESC_Brake_Effort"
  Runnable_IMAP_10ms_sys/72(IMAPve_g_EMS_Engine_Speed) -> BusCreator/72  "IMAPve_g_EMS_Engine_Speed"
  Runnable_IMAP_10ms_sys/73(IMAPve_d_ESC_Veh_Standstill) -> BusCreator/73  "IMAPve_d_ESC_Veh_Standstill"
  Runnable_IMAP_10ms_sys/74(IMAPve_d_TCU_Actual_Gear) -> BusCreator/74  "IMAPve_d_TCU_Actual_Gear"
  Runnable_IMAP_10ms_sys/75(IMAPve_d_TCU_Target_Gear) -> BusCreator/75  "IMAPve_d_TCU_Target_Gear"
  Runnable_IMAP_10ms_sys/76(IMAPve_d_TCU_PRND_State) -> BusCreator/76  "IMAPve_d_TCU_PRND_State"
  Runnable_IMAP_10ms_sys/77(IMAPve_d_BCM_Ignition_State) -> BusCreator/77  "IMAPve_d_BCM_Ignition_State"
  Runnable_IMAP_10ms_sys/78(IMAPve_d_ACU_Driver_Belt) -> BusCreator/78  "IMAPve_d_ACU_Driver_Belt"
  Runnable_IMAP_10ms_sys/79(IMAPve_d_SWS_Failure_Status) -> BusCreator/79  "IMAPve_d_SWS_Failure_Status"
  Runnable_IMAP_10ms_sys/80(IMAPve_d_ESC_OFF) -> BusCreator/80  "IMAPve_d_ESC_OFF"
  Runnable_IMAP_10ms_sys/81(IMAPve_d_ESC_AlarmSig) -> BusCreator/81  "IMAPve_d_ESC_AlarmSig"
  Runnable_IMAP_10ms_sys/82(IMAPve_d_ESC_ESC_Active) -> BusCreator/82  "IMAPve_d_ESC_ESC_Active"
  Runnable_IMAP_10ms_sys/83(IMAPve_d_ESC_MSR_Active) -> BusCreator/83  "IMAPve_d_ESC_MSR_Active"
  Runnable_IMAP_10ms_sys/84(IMAPve_d_ESC_TCS_Active) -> BusCreator/84  "IMAPve_d_ESC_TCS_Active"
  Runnable_IMAP_10ms_sys/85(IMAPve_d_ESC_VehSpd_Valid) -> BusCreator/85  "IMAPve_d_ESC_VehSpd_Valid"
  Runnable_IMAP_10ms_sys/86(IMAPve_d_ESC_ABS_Active) -> BusCreator/86  "IMAPve_d_ESC_ABS_Active"
  Runnable_IMAP_10ms_sys/87(IMAPve_d_ESC_ABS_Valid) -> BusCreator/87  "IMAPve_d_ESC_ABS_Valid"
  Runnable_IMAP_10ms_sys/88(IMAPve_d_ESC_ABS_AlarmSig) -> BusCreator/88  "IMAPve_d_ESC_ABS_AlarmSig"
  Runnable_IMAP_10ms_sys/89(IMAPve_d_ESC_FL_WheelPulVal) -> BusCreator/89  "IMAPve_d_ESC_FL_WheelPulVal"
  Runnable_IMAP_10ms_sys/90(IMAPve_d_ESC_FR_WheelPulVal) -> BusCreator/90  "IMAPve_d_ESC_FR_WheelPulVal"
  Runnable_IMAP_10ms_sys/91(IMAPve_d_ESC_RL_WheelPulVal) -> BusCreator/91  "IMAPve_d_ESC_RL_WheelPulVal"
  Runnable_IMAP_10ms_sys/92(IMAPve_d_ESC_RR_WheelPulVal) -> BusCreator/92  "IMAPve_d_ESC_RR_WheelPulVal"
  Runnable_IMAP_10ms_sys/93(IMAPve_g_ESC_FL_WhlSpd) -> BusCreator/93  "IMAPve_g_ESC_FL_WhlSpd"
  Runnable_IMAP_10ms_sys/94(IMAPve_d_ESC_FL_WhlSpd_Fault) -> BusCreator/94  "IMAPve_d_ESC_FL_WhlSpd_Fault"
  Runnable_IMAP_10ms_sys/95(IMAPve_g_ESC_FR_WhlSpd) -> BusCreator/95  "IMAPve_g_ESC_FR_WhlSpd"
  Runnable_IMAP_10ms_sys/96(IMAPve_d_ESC_FR_WhlSpd_Fault) -> BusCreator/96  "IMAPve_d_ESC_FR_WhlSpd_Fault"
  Runnable_IMAP_10ms_sys/97(IMAPve_g_ESC_RL_WhlSpd) -> BusCreator/97  "IMAPve_g_ESC_RL_WhlSpd"
  Runnable_IMAP_10ms_sys/98(IMAPve_d_ESC_RL_WhlSpd_Fault) -> BusCreator/98  "IMAPve_d_ESC_RL_WhlSpd_Fault"
  Runnable_IMAP_10ms_sys/99(IMAPve_g_ESC_RR_WhlSpd) -> BusCreator/99  "IMAPve_g_ESC_RR_WhlSpd"
  Runnable_IMAP_10ms_sys/100(IMAPve_d_ESC_RR_WhlSpd_Fault) -> BusCreator/100  "IMAPve_d_ESC_RR_WhlSpd_Fault"
  Runnable_IMAP_10ms_sys/101(IMAPve_d_ESC_FL_Wheel_Pulse) -> BusCreator/101  "IMAPve_d_ESC_FL_Wheel_Pulse"
  Runnable_IMAP_10ms_sys/102(IMAPve_d_ESC_FR_Wheel_Pulse) -> BusCreator/102  "IMAPve_d_ESC_FR_Wheel_Pulse"
  Runnable_IMAP_10ms_sys/103(IMAPve_d_ESC_RL_Wheel_Pulse) -> BusCreator/103  "IMAPve_d_ESC_RL_Wheel_Pulse"
  Runnable_IMAP_10ms_sys/104(IMAPve_d_ESC_RR_Wheel_Pulse) -> BusCreator/104  "IMAPve_d_ESC_RR_Wheel_Pulse"
  Runnable_IMAP_10ms_sys/105(IMAPve_d_TCU_AT_Failure) -> BusCreator/105  "IMAPve_d_TCU_AT_Failure"
  Runnable_IMAP_10ms_sys/106(IMAPve_d_TCU_Shift_Valid) -> BusCreator/106  "IMAPve_d_TCU_Shift_Valid"
  Runnable_IMAP_10ms_sys/107(IMAPve_d_TCU_DCT_Clutch_State) -> BusCreator/107  "IMAPve_d_TCU_DCT_Clutch_State"
  Runnable_IMAP_10ms_sys/108(IMAPve_d_TCU_Gear_Engage) -> BusCreator/108  "IMAPve_d_TCU_Gear_Engage"
  Runnable_IMAP_10ms_sys/109(IMAPve_d_TCU_Select_ATMode) -> BusCreator/109  "IMAPve_d_TCU_Select_ATMode"
  Runnable_IMAP_10ms_sys/110(IMAPve_d_EMS_Engine_Status) -> BusCreator/110  "IMAPve_d_EMS_Engine_Status"
  Runnable_IMAP_10ms_sys/111(IMAPve_d_EMS_Gearbox_CtlAvail) -> BusCreator/111  "IMAPve_d_EMS_Gearbox_CtlAvail"
  Runnable_IMAP_10ms_sys/112(IMAPve_d_ESC_Brake_Failsafe) -> BusCreator/112  "IMAPve_d_ESC_Brake_Failsafe"
  Runnable_IMAP_10ms_sys/113(IMAPve_d_ESC_AEB_Available) -> BusCreator/113  "IMAPve_d_ESC_AEB_Available"
  Runnable_IMAP_10ms_sys/114(IMAPve_d_ESC_AEB_Active) -> BusCreator/114  "IMAPve_d_ESC_AEB_Active"
  Runnable_IMAP_10ms_sys/115(IMAPve_d_ESC_ACC_Available) -> BusCreator/115  "IMAPve_d_ESC_ACC_Available"
  Runnable_IMAP_10ms_sys/116(IMAPve_d_ESC_ACC_Active) -> BusCreator/116  "IMAPve_d_ESC_ACC_Active"
  Runnable_IMAP_10ms_sys/117(IMAPve_d_EMS_ACC_Effective) -> BusCreator/117  "IMAPve_d_EMS_ACC_Effective"
  Runnable_IMAP_10ms_sys/118(IMAPve_d_BCM_FrontWiper_State) -> BusCreator/118  "IMAPve_d_BCM_FrontWiper_State"
  Runnable_IMAP_10ms_sys/119(IMAPve_d_BCM_CHMSL_Status) -> BusCreator/119  "IMAPve_d_BCM_CHMSL_Status"
  Runnable_IMAP_10ms_sys/120(IMAPve_d_BCM_BrakeLamp_State) -> BusCreator/120  "IMAPve_d_BCM_BrakeLamp_State"
  Runnable_IMAP_10ms_sys/121(IMAPve_d_ACU_Passenger_Belt) -> BusCreator/121  "IMAPve_d_ACU_Passenger_Belt"
  Runnable_IMAP_10ms_sys/122(IMAPve_d_EMS_ACC_CtlAvail) -> BusCreator/122  "IMAPve_d_EMS_ACC_CtlAvail"
  Runnable_IMAP_10ms_sys/123(IMAPve_d_EMS_ACC_Inhibited) -> BusCreator/123  "IMAPve_d_EMS_ACC_Inhibited"
  Runnable_IMAP_10ms_sys/124(IMAPve_d_EMS_Brake_Pedal) -> BusCreator/124  "IMAPve_d_EMS_Brake_Pedal"
  Runnable_IMAP_10ms_sys/125(IMAPve_d_BCM_LowBeam_State) -> BusCreator/125  "IMAPve_d_BCM_LowBeam_State"
  Runnable_IMAP_10ms_sys/126(IMAPve_d_BCM_HighBeam_State) -> BusCreator/126  "IMAPve_d_BCM_HighBeam_State"
  Runnable_IMAP_10ms_sys/127(IMAPve_d_EPB_Status) -> BusCreator/127  "IMAPve_d_EPB_Status"
  Runnable_IMAP_10ms_sys/128(IMAPve_d_EPB_Display_Req) -> BusCreator/128  "IMAPve_d_EPB_Display_Req"
  Runnable_IMAP_10ms_sys/129(IMAPve_d_EPB_Warn_Req) -> BusCreator/129  "IMAPve_d_EPB_Warn_Req"
  Runnable_IMAP_10ms_sys/130(IMAPve_d_EPB_Switch_State) -> BusCreator/130  "IMAPve_d_EPB_Switch_State"
  Runnable_IMAP_10ms_sys/131(IMAPve_d_EPB_Switch_Valid) -> BusCreator/131  "IMAPve_d_EPB_Switch_Valid"
  Runnable_IMAP_10ms_sys/132(IMAPve_d_ESC_Drive_Direction) -> BusCreator/132  "IMAPve_d_ESC_Drive_Direction"
  Runnable_IMAP_10ms_sys/133(IMAPve_d_ESC_Hold_State) -> BusCreator/133  "IMAPve_d_ESC_Hold_State"
  Runnable_IMAP_10ms_sys/134(IMAPve_d_EPS_Steer_Hold_State) -> BusCreator/134  "IMAPve_d_EPS_Steer_Hold_State"
  Runnable_IMAP_10ms_sys/135(IMAPve_d_EPS_Warning_State) -> BusCreator/135  "IMAPve_d_EPS_Warning_State"
  Runnable_IMAP_10ms_sys/136(IMAPve_g_EPS_PowerCon) -> BusCreator/136  "IMAPve_g_EPS_PowerCon"
  Runnable_IMAP_10ms_sys/137(IMAPve_d_ESC_EBD_AlarmSig) -> BusCreator/137  "IMAPve_d_ESC_EBD_AlarmSig"
  Runnable_IMAP_10ms_sys/138(IMAPve_d_ESC_AVH_Status) -> BusCreator/138  "IMAPve_d_ESC_AVH_Status"
  Runnable_IMAP_10ms_sys/139(IMAPve_g_BCM_Battery_Voltage) -> BusCreator/139  "IMAPve_g_BCM_Battery_Voltage"
  Runnable_IMAP_10ms_sys/140(IMAPve_d_TBOX_LocalTimeY) -> BusCreator/140  "IMAPve_d_TBOX_LocalTimeY"
  Runnable_IMAP_10ms_sys/141(IMAPve_d_TBOX_LocalTimeM) -> BusCreator/141  "IMAPve_d_TBOX_LocalTimeM"
  Runnable_IMAP_10ms_sys/142(IMAPve_d_TBOX_LocalTimeD) -> BusCreator/142  "IMAPve_d_TBOX_LocalTimeD"
  Runnable_IMAP_10ms_sys/143(IMAPve_d_TBOX_LocalTimeH) -> BusCreator/143  "IMAPve_d_TBOX_LocalTimeH"
  Runnable_IMAP_10ms_sys/144(IMAPve_d_TBOX_LocalTimeMin) -> BusCreator/144  "IMAPve_d_TBOX_LocalTimeMin"
  Runnable_IMAP_10ms_sys/145(IMAPve_d_TBOX_LocalTimeS) -> BusCreator/145  "IMAPve_d_TBOX_LocalTimeS"
  Runnable_IMAP_10ms_sys/146(IMAPve_d_TBOX_LocalTime_Valid) -> BusCreator/146  "IMAPve_d_TBOX_LocalTime_Valid"
  Runnable_IMAP_10ms_sys/147(IMAPve_d_Radar_State) -> BusCreator/147  "IMAPve_d_Radar_State"
  Runnable_IMAP_10ms_sys/148(IMAPve_d_Time_System_Clock) -> BusCreator/148  "IMAPve_d_Time_System_Clock"
  Runnable_IMAP_10ms_sys/149(IMAPve_g_GW_IC_Odometer) -> BusCreator/149  "IMAPve_g_GW_IC_Odometer"
  Runnable_IMAP_10ms_sys/150(IMAPve_d_Outside_Temp) -> BusCreator/150  "IMAPve_d_Outside_Temp"
  Runnable_IMAP_10ms_sys/151(IMAPve_d_ORI_CIPV_ID) -> BusCreator/151  "IMAPve_d_ORI_CIPV_ID"
  Runnable_IMAP_10ms_sys/152(IMAPve_d_ORI_Obj_Num) -> BusCreator/152  "IMAPve_d_ORI_Obj_Num"
  Runnable_IMAP_10ms_sys/153(IMAPva_d_ORI_Obj_Class) -> BusCreator/153  "IMAPva_d_ORI_Obj_Class"
  Runnable_IMAP_10ms_sys/154(IMAPva_g_ORI_Obj_RelVel) -> BusCreator/154  "IMAPva_g_ORI_Obj_RelVel"
  Runnable_IMAP_10ms_sys/155(IMAPva_g_ORI_Obj_LongDis) -> BusCreator/155  "IMAPva_g_ORI_Obj_LongDis"
  Runnable_IMAP_10ms_sys/156(IMAPva_g_ORI_Obj_LAngle) -> BusCreator/156  "IMAPva_g_ORI_Obj_LAngle"
  Runnable_IMAP_10ms_sys/157(IMAPva_g_ORI_Obj_RAngle) -> BusCreator/157  "IMAPva_g_ORI_Obj_RAngle"
  Runnable_IMAP_10ms_sys/158(IMAPva_g_ORI_Obj_Width) -> BusCreator/158  "IMAPva_g_ORI_Obj_Width"
  Runnable_IMAP_10ms_sys/159(IMAPva_d_ORI_Obj_ID) -> BusCreator/159  "IMAPva_d_ORI_Obj_ID"
  Runnable_IMAP_10ms_sys/160(IMAPve_g_ORI_L0_C3) -> BusCreator/160  "IMAPve_g_ORI_L0_C3"
  Runnable_IMAP_10ms_sys/161(IMAPve_g_ORI_L0_C2) -> BusCreator/161  "IMAPve_g_ORI_L0_C2"
  Runnable_IMAP_10ms_sys/162(IMAPve_g_ORI_L0_C1) -> BusCreator/162  "IMAPve_g_ORI_L0_C1"
  Runnable_IMAP_10ms_sys/163(IMAPve_g_ORI_L0_C0) -> BusCreator/163  "IMAPve_g_ORI_L0_C0"
  Runnable_IMAP_10ms_sys/164(IMAPve_d_ORI_L0_Type) -> BusCreator/164  "IMAPve_d_ORI_L0_Type"
  Runnable_IMAP_10ms_sys/165(IMAPve_g_ORI_L0_VR) -> BusCreator/165  "IMAPve_g_ORI_L0_VR"
  Runnable_IMAP_10ms_sys/166(IMAPve_g_ORI_L0_W) -> BusCreator/166  "IMAPve_g_ORI_L0_W"
  Runnable_IMAP_10ms_sys/167(IMAPve_g_ORI_L1_C3) -> BusCreator/167  "IMAPve_g_ORI_L1_C3"
  Runnable_IMAP_10ms_sys/168(IMAPve_g_ORI_L1_C2) -> BusCreator/168  "IMAPve_g_ORI_L1_C2"
  Runnable_IMAP_10ms_sys/169(IMAPve_g_ORI_L1_C1) -> BusCreator/169  "IMAPve_g_ORI_L1_C1"
  Runnable_IMAP_10ms_sys/170(IMAPve_g_ORI_L1_C0) -> BusCreator/170  "IMAPve_g_ORI_L1_C0"
  Runnable_IMAP_10ms_sys/171(IMAPve_d_ORI_L1_Type) -> BusCreator/171  "IMAPve_d_ORI_L1_Type"
  Runnable_IMAP_10ms_sys/172(IMAPve_g_ORI_L1_VR) -> BusCreator/172  "IMAPve_g_ORI_L1_VR"
  Runnable_IMAP_10ms_sys/173(IMAPve_g_ORI_L1_W) -> BusCreator/173  "IMAPve_g_ORI_L1_W"
  Runnable_IMAP_10ms_sys/174(IMAPve_g_ORI_R0_C3) -> BusCreator/174  "IMAPve_g_ORI_R0_C3"
  Runnable_IMAP_10ms_sys/175(IMAPve_g_ORI_R0_C2) -> BusCreator/175  "IMAPve_g_ORI_R0_C2"
  Runnable_IMAP_10ms_sys/176(IMAPve_g_ORI_R0_C1) -> BusCreator/176  "IMAPve_g_ORI_R0_C1"
  Runnable_IMAP_10ms_sys/177(IMAPve_g_ORI_R0_C0) -> BusCreator/177  "IMAPve_g_ORI_R0_C0"
  Runnable_IMAP_10ms_sys/178(IMAPve_d_ORI_R0_LT) -> BusCreator/178  "IMAPve_d_ORI_R0_LT"
  Runnable_IMAP_10ms_sys/179(IMAPve_g_ORI_R0_VR) -> BusCreator/179  "IMAPve_g_ORI_R0_VR"
  Runnable_IMAP_10ms_sys/180(IMAPve_g_ORI_R0_W) -> BusCreator/180  "IMAPve_g_ORI_R0_W"
  Runnable_IMAP_10ms_sys/181(IMAPve_g_ORI_R1_C3) -> BusCreator/181  "IMAPve_g_ORI_R1_C3"
  Runnable_IMAP_10ms_sys/182(IMAPve_g_ORI_R1_C2) -> BusCreator/182  "IMAPve_g_ORI_R1_C2"
  Runnable_IMAP_10ms_sys/183(IMAPve_g_ORI_R1_C1) -> BusCreator/183  "IMAPve_g_ORI_R1_C1"
  Runnable_IMAP_10ms_sys/184(IMAPve_g_ORI_R1_C0) -> BusCreator/184  "IMAPve_g_ORI_R1_C0"
  Runnable_IMAP_10ms_sys/185(IMAPve_d_ORI_R1_LT) -> BusCreator/185  "IMAPve_d_ORI_R1_LT"
  Runnable_IMAP_10ms_sys/186(IMAPve_g_ORI_R1_VR) -> BusCreator/186  "IMAPve_g_ORI_R1_VR"
  Runnable_IMAP_10ms_sys/187(IMAPve_g_ORI_R1_W) -> BusCreator/187  "IMAPve_g_ORI_R1_W"
  Runnable_IMAP_10ms_sys/188(IMAPve_d_Sensor_Status) -> BusCreator/188  "IMAPve_d_Sensor_Status"
  Runnable_IMAP_10ms_sys/189(IMAPve_d_LF_Radar_Status) -> BusCreator/189  "IMAPve_d_LF_Radar_Status"
  Runnable_IMAP_10ms_sys/190(IMAPve_d_RF_Radar_Status) -> BusCreator/190  "IMAPve_d_RF_Radar_Status"
  Runnable_IMAP_10ms_sys/191(IMAPve_d_LR_Radar_Status) -> BusCreator/191  "IMAPve_d_LR_Radar_Status"
  Runnable_IMAP_10ms_sys/192(IMAPve_d_RR_Radar_Status) -> BusCreator/192  "IMAPve_d_RR_Radar_Status"
  Runnable_IMAP_10ms_sys/193(IMAPve_d_Fusion_Status) -> BusCreator/193  "IMAPve_d_Fusion_Status"
  Runnable_IMAP_10ms_sys/194(IMAPve_d_Fusion_Time_Stamp) -> BusCreator/194  "IMAPve_d_Fusion_Time_Stamp"
  Runnable_IMAP_10ms_sys/195(IMAPve_d_obj_Num) -> BusCreator/195  "IMAPve_d_obj_Num"
  Runnable_IMAP_10ms_sys/196(IMAPva_d_obj_id) -> BusCreator/196  "IMAPva_d_obj_id"
  Runnable_IMAP_10ms_sys/197(IMAPva_g_obj_pos_x) -> BusCreator/197  "IMAPva_g_obj_pos_x"
  Runnable_IMAP_10ms_sys/198(IMAPva_g_obj_pos_y) -> BusCreator/198  "IMAPva_g_obj_pos_y"
  Runnable_IMAP_10ms_sys/199(IMAPva_g_obj_vel_x) -> BusCreator/199  "IMAPva_g_obj_vel_x"
  Runnable_IMAP_10ms_sys/200(IMAPva_g_obj_vel_y) -> BusCreator/200  "IMAPva_g_obj_vel_y"
  Runnable_IMAP_10ms_sys/201(IMAPva_g_obj_acc_x) -> BusCreator/201  "IMAPva_g_obj_acc_x"
  Runnable_IMAP_10ms_sys/202(IMAPva_g_obj_acc_y) -> BusCreator/202  "IMAPva_g_obj_acc_y"
  Runnable_IMAP_10ms_sys/203(IMAPva_g_obj_pos_var_x) -> BusCreator/203  "IMAPva_g_obj_pos_var_x"
  Runnable_IMAP_10ms_sys/204(IMAPva_g_obj_pos_var_y) -> BusCreator/204  "IMAPva_g_obj_pos_var_y"
  Runnable_IMAP_10ms_sys/205(IMAPva_g_obj_pos_var_xy) -> BusCreator/205  "IMAPva_g_obj_pos_var_xy"
  Runnable_IMAP_10ms_sys/206(IMAPva_g_obj_width) -> BusCreator/206  "IMAPva_g_obj_width"
  Runnable_IMAP_10ms_sys/207(IMAPva_g_obj_length) -> BusCreator/207  "IMAPva_g_obj_length"
  Runnable_IMAP_10ms_sys/208(IMAPva_d_obj_class) -> BusCreator/208  "IMAPva_d_obj_class"
  Runnable_IMAP_10ms_sys/209(IMAPva_d_obj_lane) -> BusCreator/209  "IMAPva_d_obj_lane"
  Runnable_IMAP_10ms_sys/210(IMAPva_d_obj_status) -> BusCreator/210  "IMAPva_d_obj_status"
  Runnable_IMAP_10ms_sys/211(IMAPva_d_obj_age) -> BusCreator/211  "IMAPva_d_obj_age"
  Runnable_IMAP_10ms_sys/212(IMAPva_d_obj_TurnLight) -> BusCreator/212  "IMAPva_d_obj_TurnLight"
  Runnable_IMAP_10ms_sys/213(IMAPva_d_obj_BrakeLight) -> BusCreator/213  "IMAPva_d_obj_BrakeLight"
  Runnable_IMAP_10ms_sys/214(IMAPva_d_obj_MotionStatus) -> BusCreator/214  "IMAPva_d_obj_MotionStatus"
  Runnable_IMAP_10ms_sys/215(IMAPve_d_Road_Type) -> BusCreator/215  "IMAPve_d_Road_Type"
  Runnable_IMAP_10ms_sys/216(IMAPve_g_L0_C0) -> BusCreator/216  "IMAPve_g_L0_C0"
  Runnable_IMAP_10ms_sys/217(IMAPve_g_L0_C1) -> BusCreator/217  "IMAPve_g_L0_C1"
  Runnable_IMAP_10ms_sys/218(IMAPve_g_L0_C2) -> BusCreator/218  "IMAPve_g_L0_C2"
  Runnable_IMAP_10ms_sys/219(IMAPve_g_L0_C3) -> BusCreator/219  "IMAPve_g_L0_C3"
  Runnable_IMAP_10ms_sys/220(IMAPve_g_L0_VR) -> BusCreator/220  "IMAPve_g_L0_VR"
  Runnable_IMAP_10ms_sys/221(IMAPve_d_L0_Q) -> BusCreator/221  "IMAPve_d_L0_Q"
  Runnable_IMAP_10ms_sys/222(IMAPve_d_L0_Type) -> BusCreator/222  "IMAPve_d_L0_Type"
  Runnable_IMAP_10ms_sys/223(IMAPve_g_L0_W) -> BusCreator/223  "IMAPve_g_L0_W"
  Runnable_IMAP_10ms_sys/224(IMAPve_g_R0_C0) -> BusCreator/224  "IMAPve_g_R0_C0"
  Runnable_IMAP_10ms_sys/225(IMAPve_g_R0_C1) -> BusCreator/225  "IMAPve_g_R0_C1"
  Runnable_IMAP_10ms_sys/226(IMAPve_g_R0_C2) -> BusCreator/226  "IMAPve_g_R0_C2"
  Runnable_IMAP_10ms_sys/227(IMAPve_g_R0_C3) -> BusCreator/227  "IMAPve_g_R0_C3"
  Runnable_IMAP_10ms_sys/228(IMAPve_g_R0_VR) -> BusCreator/228  "IMAPve_g_R0_VR"
  Runnable_IMAP_10ms_sys/229(IMAPve_d_R0_Q) -> BusCreator/229  "IMAPve_d_R0_Q"
  Runnable_IMAP_10ms_sys/230(IMAPve_d_R0_Type) -> BusCreator/230  "IMAPve_d_R0_Type"
  Runnable_IMAP_10ms_sys/231(IMAPve_g_R0_W) -> BusCreator/231  "IMAPve_g_R0_W"
  Runnable_IMAP_10ms_sys/232(IMAPve_g_L1_C0) -> BusCreator/232  "IMAPve_g_L1_C0"
  Runnable_IMAP_10ms_sys/233(IMAPve_g_L1_C1) -> BusCreator/233  "IMAPve_g_L1_C1"
  Runnable_IMAP_10ms_sys/234(IMAPve_g_L1_C2) -> BusCreator/234  "IMAPve_g_L1_C2"
  Runnable_IMAP_10ms_sys/235(IMAPve_g_L1_C3) -> BusCreator/235  "IMAPve_g_L1_C3"
  Runnable_IMAP_10ms_sys/236(IMAPve_g_L1_VR) -> BusCreator/236  "IMAPve_g_L1_VR"
  Runnable_IMAP_10ms_sys/237(IMAPve_d_L1_Q) -> BusCreator/237  "IMAPve_d_L1_Q"
  Runnable_IMAP_10ms_sys/238(IMAPve_d_L1_Type) -> BusCreator/238  "IMAPve_d_L1_Type"
  Runnable_IMAP_10ms_sys/239(IMAPve_g_L1_W) -> BusCreator/239  "IMAPve_g_L1_W"
  Runnable_IMAP_10ms_sys/240(IMAPve_g_R1_C0) -> BusCreator/240  "IMAPve_g_R1_C0"
  Runnable_IMAP_10ms_sys/241(IMAPve_g_R1_C1) -> BusCreator/241  "IMAPve_g_R1_C1"
  Runnable_IMAP_10ms_sys/242(IMAPve_g_R1_C2) -> BusCreator/242  "IMAPve_g_R1_C2"
  Runnable_IMAP_10ms_sys/243(IMAPve_g_R1_C3) -> BusCreator/243  "IMAPve_g_R1_C3"
  Runnable_IMAP_10ms_sys/244(IMAPve_g_R1_VR) -> BusCreator/244  "IMAPve_g_R1_VR"
  Runnable_IMAP_10ms_sys/245(IMAPve_d_R1_Q) -> BusCreator/245  "IMAPve_d_R1_Q"
  Runnable_IMAP_10ms_sys/246(IMAPve_d_R1_Type) -> BusCreator/246  "IMAPve_d_R1_Type"
  Runnable_IMAP_10ms_sys/247(IMAPve_g_R1_W) -> BusCreator/247  "IMAPve_g_R1_W"
  Runnable_IMAP_10ms_sys/248(IMAPve_g_L0_C0_Back) -> BusCreator/248  "IMAPve_g_L0_C0_Back"
  Runnable_IMAP_10ms_sys/249(IMAPve_g_L0_C1_Back) -> BusCreator/249  "IMAPve_g_L0_C1_Back"
  Runnable_IMAP_10ms_sys/250(IMAPve_g_L0_C2_Back) -> BusCreator/250  "IMAPve_g_L0_C2_Back"
  Runnable_IMAP_10ms_sys/251(IMAPve_g_L0_C3_Back) -> BusCreator/251  "IMAPve_g_L0_C3_Back"
  Runnable_IMAP_10ms_sys/252(IMAPve_g_L0_Range_Back) -> BusCreator/252  "IMAPve_g_L0_Range_Back"
  Runnable_IMAP_10ms_sys/253(IMAPve_g_R0_C0_Back) -> BusCreator/253  "IMAPve_g_R0_C0_Back"
  Runnable_IMAP_10ms_sys/254(IMAPve_g_R0_C1_Back) -> BusCreator/254  "IMAPve_g_R0_C1_Back"
  Runnable_IMAP_10ms_sys/255(IMAPve_g_R0_C2_Back) -> BusCreator/255  "IMAPve_g_R0_C2_Back"
  Runnable_IMAP_10ms_sys/256(IMAPve_g_R0_C3_Back) -> BusCreator/256  "IMAPve_g_R0_C3_Back"
  Runnable_IMAP_10ms_sys/257(IMAPve_g_R0_Range_Back) -> BusCreator/257  "IMAPve_g_R0_Range_Back"
  Runnable_IMAP_10ms_sys/258(IMAPve_g_L1_C0_Back) -> BusCreator/258  "IMAPve_g_L1_C0_Back"
  Runnable_IMAP_10ms_sys/259(IMAPve_g_L1_C1_Back) -> BusCreator/259  "IMAPve_g_L1_C1_Back"
  Runnable_IMAP_10ms_sys/260(IMAPve_g_L1_C2_Back) -> BusCreator/260  "IMAPve_g_L1_C2_Back"
  Runnable_IMAP_10ms_sys/261(IMAPve_g_L1_C3_Back) -> BusCreator/261  "IMAPve_g_L1_C3_Back"
  Runnable_IMAP_10ms_sys/262(IMAPve_g_L1_Range_Back) -> BusCreator/262  "IMAPve_g_L1_Range_Back"
  Runnable_IMAP_10ms_sys/263(IMAPve_g_R1_C0_Back) -> BusCreator/263  "IMAPve_g_R1_C0_Back"
  Runnable_IMAP_10ms_sys/264(IMAPve_g_R1_C1_Back) -> BusCreator/264  "IMAPve_g_R1_C1_Back"
  Runnable_IMAP_10ms_sys/265(IMAPve_g_R1_C2_Back) -> BusCreator/265  "IMAPve_g_R1_C2_Back"
  Runnable_IMAP_10ms_sys/266(IMAPve_g_R1_C3_Back) -> BusCreator/266  "IMAPve_g_R1_C3_Back"
  Runnable_IMAP_10ms_sys/267(IMAPve_g_R1_Range_Back) -> BusCreator/267  "IMAPve_g_R1_Range_Back"
  Runnable_IMAP_10ms_sys/268(IMAPve_g_Lrg_C0_BACK) -> BusCreator/268  "IMAPve_g_Lrg_C0_BACK"
  Runnable_IMAP_10ms_sys/269(IMAPve_g_Lrg_C1_BACK) -> BusCreator/269  "IMAPve_g_Lrg_C1_BACK"
  Runnable_IMAP_10ms_sys/270(IMAPve_g_Lrg_C2_BACK) -> BusCreator/270  "IMAPve_g_Lrg_C2_BACK"
  Runnable_IMAP_10ms_sys/271(IMAPve_g_Lrg_C3_BACK) -> BusCreator/271  "IMAPve_g_Lrg_C3_BACK"
  Runnable_IMAP_10ms_sys/272(IMAPve_g_Lrg_VR_Start_BACK) -> BusCreator/272  "IMAPve_g_Lrg_VR_Start_BACK"
  Runnable_IMAP_10ms_sys/273(IMAPve_g_Lrg_VR_End_BACK) -> BusCreator/273  "IMAPve_g_Lrg_VR_End_BACK"
  Runnable_IMAP_10ms_sys/274(IMAPve_d_Lrg_Q_BACK) -> BusCreator/274  "IMAPve_d_Lrg_Q_BACK"
  Runnable_IMAP_10ms_sys/275(IMAPve_d_Lrg_TYPE_BACK) -> BusCreator/275  "IMAPve_d_Lrg_TYPE_BACK"
  Runnable_IMAP_10ms_sys/276(IMAPve_g_Rrg_C0_BACK) -> BusCreator/276  "IMAPve_g_Rrg_C0_BACK"
  Runnable_IMAP_10ms_sys/277(IMAPve_g_Rrg_C1_BACK) -> BusCreator/277  "IMAPve_g_Rrg_C1_BACK"
  Runnable_IMAP_10ms_sys/278(IMAPve_g_Rrg_C2_BACK) -> BusCreator/278  "IMAPve_g_Rrg_C2_BACK"
  Runnable_IMAP_10ms_sys/279(IMAPve_g_Rrg_C3_BACK) -> BusCreator/279  "IMAPve_g_Rrg_C3_BACK"
  Runnable_IMAP_10ms_sys/280(IMAPve_g_Rrg_VR_Start_BACK) -> BusCreator/280  "IMAPve_g_Rrg_VR_Start_BACK"
  Runnable_IMAP_10ms_sys/281(IMAPve_g_Rrg_VR_End_BACK) -> BusCreator/281  "IMAPve_g_Rrg_VR_End_BACK"
  Runnable_IMAP_10ms_sys/282(IMAPve_d_Rrg_Q_BACK) -> BusCreator/282  "IMAPve_d_Rrg_Q_BACK"
  Runnable_IMAP_10ms_sys/283(IMAPve_d_Rrg_TYPE_BACK) -> BusCreator/283  "IMAPve_d_Rrg_TYPE_BACK"
  Runnable_IMAP_10ms_sys/284(IMAPve_d_Sign_ISA_Value) -> BusCreator/284  "IMAPve_d_Sign_ISA_Value"
  Runnable_IMAP_10ms_sys/285(IMAPve_d_ISA_Popup_Message) -> BusCreator/285  "IMAPve_d_ISA_Popup_Message"
  Runnable_IMAP_10ms_sys/286(IMAPve_d_ISA_Sign_Type) -> BusCreator/286  "IMAPve_d_ISA_Sign_Type"
  Runnable_IMAP_10ms_sys/287(IMAPve_d_ISA_Status) -> BusCreator/287  "IMAPve_d_ISA_Status"
  Runnable_IMAP_10ms_sys/288(IMAPve_d_TSR_Sign_Type) -> BusCreator/288  "IMAPve_d_TSR_Sign_Type"
  Runnable_IMAP_10ms_sys/289(IMAPve_g_Camera_Signal_Fault) -> BusCreator/289  "IMAPve_g_Camera_Signal_Fault"
  Runnable_IMAP_10ms_sys/290(IMAPve_d_Camera_State) -> BusCreator/290  "IMAPve_d_Camera_State"
  Runnable_IMAP_10ms_sys/291(IMAPve_d_Radar_FaultBitSetting_Signal) -> BusCreator/291  "IMAPve_d_Radar_FaultBitSetting_Signal"
  Runnable_IMAP_10ms_sys/292(IMAPve_d_Camera_Status) -> BusCreator/292  "IMAPve_d_Camera_Status"
  Runnable_IMAP_10ms_sys/293(IMAPve_d_ESC_FLW_Direction) -> BusCreator/293  "IMAPve_d_ESC_FLW_Direction"
  Runnable_IMAP_10ms_sys/294(IMAPve_d_ESC_FRW_Direction) -> BusCreator/294  "IMAPve_d_ESC_FRW_Direction"
  Runnable_IMAP_10ms_sys/295(IMAPve_d_ESC_TCS_ErrorStatus) -> BusCreator/295  "IMAPve_d_ESC_TCS_ErrorStatus"
  Runnable_IMAP_10ms_sys/296(IMAPve_d_ESC_RLW_Direction) -> BusCreator/296  "IMAPve_d_ESC_RLW_Direction"
  Runnable_IMAP_10ms_sys/297(IMAPve_d_ESC_RRW_Direction) -> BusCreator/297  "IMAPve_d_ESC_RRW_Direction"
  Runnable_IMAP_10ms_sys/298(IMAPve_d_ESC_EPB_ErrorStatus) -> BusCreator/298  "IMAPve_d_ESC_EPB_ErrorStatus"
  Runnable_IMAP_10ms_sys/299(IMAPve_d_EPS_SteeringAngle_Flag) -> BusCreator/299  "IMAPve_d_EPS_SteeringAngle_Flag"
  Runnable_IMAP_10ms_sys/300(IMAPve_g_EPS_SteeringAngle) -> BusCreator/300  "IMAPve_g_EPS_SteeringAngle"
  Runnable_IMAP_10ms_sys/301(IMAPve_d_EPS_Driver_Override) -> BusCreator/301  "IMAPve_d_EPS_Driver_Override"
  Runnable_IMAP_10ms_sys/302(IMAPve_d_EPS_Driver_Active_ESA) -> BusCreator/302  "IMAPve_d_EPS_Driver_Active_ESA"
  Runnable_IMAP_10ms_sys/303(IMAPve_d_EPS_ESA_State) -> BusCreator/303  "IMAPve_d_EPS_ESA_State"
  Runnable_IMAP_10ms_sys/304(IMAPve_d_ACU_RearLeft_Belt) -> BusCreator/304  "IMAPve_d_ACU_RearLeft_Belt"
  Runnable_IMAP_10ms_sys/305(IMAPve_d_ACU_RearMiddle_Belt) -> BusCreator/305  "IMAPve_d_ACU_RearMiddle_Belt"
  Runnable_IMAP_10ms_sys/306(IMAPve_d_ACU_RearRight_Belt) -> BusCreator/306  "IMAPve_d_ACU_RearRight_Belt"
  Runnable_IMAP_10ms_sys/307(IMAPve_d_EMS_PowertrainCtl_State) -> BusCreator/307  "IMAPve_d_EMS_PowertrainCtl_State"
  Runnable_IMAP_10ms_sys/308(IMAPve_d_TCU_TCU_Available) -> BusCreator/308  "IMAPve_d_TCU_TCU_Available"
  Runnable_IMAP_10ms_sys/309(IMAPve_d_BCM_LeftTurn_Switch) -> BusCreator/309  "IMAPve_d_BCM_LeftTurn_Switch"
  Runnable_IMAP_10ms_sys/310(IMAPve_d_BCM_RightTurn_Switch) -> BusCreator/310  "IMAPve_d_BCM_RightTurn_Switch"
  Runnable_IMAP_10ms_sys/311(IMAPve_d_BCM_FrontWiper_Switch) -> BusCreator/311  "IMAPve_d_BCM_FrontWiper_Switch"
  Runnable_IMAP_10ms_sys/312(IMAPve_d_BCM_IHBC_Enabled) -> BusCreator/312  "IMAPve_d_BCM_IHBC_Enabled"
  Runnable_IMAP_10ms_sys/313(IMAPve_d_MP5_Work_State) -> BusCreator/313  "IMAPve_d_MP5_Work_State"
  Runnable_IMAP_10ms_sys/314(IMAPve_d_MP5_APA_ModeSelect) -> BusCreator/314  "IMAPve_d_MP5_APA_ModeSelect"
  Runnable_IMAP_10ms_sys/315(IMAPve_d_MP5_LanguageSet) -> BusCreator/315  "IMAPve_d_MP5_LanguageSet"
  Runnable_IMAP_10ms_sys/316(IMAPve_d_MP5_UPA_Switch) -> BusCreator/316  "IMAPve_d_MP5_UPA_Switch"
  Runnable_IMAP_10ms_sys/317(IMAPve_d_MP5_FLK_Activation) -> BusCreator/317  "IMAPve_d_MP5_FLK_Activation"
  Runnable_IMAP_10ms_sys/318(IMAPve_d_MP5_AutoPilot_Switch) -> BusCreator/318  "IMAPve_d_MP5_AutoPilot_Switch"
  Runnable_IMAP_10ms_sys/319(IMAPve_d_MP5_DMS_MessageType) -> BusCreator/319  "IMAPve_d_MP5_DMS_MessageType"
  Runnable_IMAP_10ms_sys/320(IMAPve_d_MP5_DMS_SystemEnable) -> BusCreator/320  "IMAPve_d_MP5_DMS_SystemEnable"
  Runnable_IMAP_10ms_sys/321(IMAPve_d_MP5_DMS_DelUserNum) -> BusCreator/321  "IMAPve_d_MP5_DMS_DelUserNum"
  Runnable_IMAP_10ms_sys/322(IMAPve_d_MP5_DMS_Sensity) -> BusCreator/322  "IMAPve_d_MP5_DMS_Sensity"
  Runnable_IMAP_10ms_sys/323(IMAPve_d_MP5_DMS_EyeFatigue) -> BusCreator/323  "IMAPve_d_MP5_DMS_EyeFatigue"
  Runnable_IMAP_10ms_sys/324(IMAPve_d_MP5_DMS_LongtimeDrive) -> BusCreator/324  "IMAPve_d_MP5_DMS_LongtimeDrive"
  Runnable_IMAP_10ms_sys/325(IMAPve_d_MP5_DMS_SideView) -> BusCreator/325  "IMAPve_d_MP5_DMS_SideView"
  Runnable_IMAP_10ms_sys/326(IMAPve_d_MP5_DMS_UsingPhone) -> BusCreator/326  "IMAPve_d_MP5_DMS_UsingPhone"
  Runnable_IMAP_10ms_sys/327(IMAPve_d_MP5_DMS_Smoking) -> BusCreator/327  "IMAPve_d_MP5_DMS_Smoking"
  Runnable_IMAP_10ms_sys/328(IMAPve_d_MP5_DMS_DrinkWater) -> BusCreator/328  "IMAPve_d_MP5_DMS_DrinkWater"
  Runnable_IMAP_10ms_sys/329(IMAPve_d_MP5_DMS_UserAccount) -> BusCreator/329  "IMAPve_d_MP5_DMS_UserAccount"
  Runnable_IMAP_10ms_sys/330(IMAPve_g_ESC_BrkWhlCylinder_Pressure) -> BusCreator/330  "IMAPve_g_ESC_BrkWhlCylinder_Pressure"
  Runnable_IMAP_10ms_sys/331(IMAPva_d_ORI_Obj_TimeStamp) -> BusCreator/331  "IMAPva_d_ORI_Obj_TimeStamp"
  Runnable_IMAP_10ms_sys/332(IMAPve_d_ORI_FS_OutOfCalib) -> BusCreator/332  "IMAPve_d_ORI_FS_OutOfCalib"
  Runnable_IMAP_10ms_sys/333(IMAPve_d_ORI_FS_Rain) -> BusCreator/333  "IMAPve_d_ORI_FS_Rain"
  Runnable_IMAP_10ms_sys/334(IMAPve_d_ORI_FS_Fog) -> BusCreator/334  "IMAPve_d_ORI_FS_Fog"
  Runnable_IMAP_10ms_sys/335(IMAPve_d_ORI_FS_Splashes0) -> BusCreator/335  "IMAPve_d_ORI_FS_Splashes0"
  Runnable_IMAP_10ms_sys/336(IMAPve_d_ORI_FS_SunRay0) -> BusCreator/336  "IMAPve_d_ORI_FS_SunRay0"
  Runnable_IMAP_10ms_sys/337(IMAPve_d_ORI_FS_LowSun0) -> BusCreator/337  "IMAPve_d_ORI_FS_LowSun0"
  Runnable_IMAP_10ms_sys/338(IMAPve_d_ORI_FS_BlurImage0) -> BusCreator/338  "IMAPve_d_ORI_FS_BlurImage0"
  Runnable_IMAP_10ms_sys/339(IMAPve_d_ORI_FS_PartialBlockage0) -> BusCreator/339  "IMAPve_d_ORI_FS_PartialBlockage0"
  Runnable_IMAP_10ms_sys/340(IMAPve_d_ORI_FS_FullBlockage0) -> BusCreator/340  "IMAPve_d_ORI_FS_FullBlockage0"
  Runnable_IMAP_10ms_sys/341(IMAPve_d_ORI_FS_FrozenWindshield0) -> BusCreator/341  "IMAPve_d_ORI_FS_FrozenWindshield0"
  Runnable_IMAP_10ms_sys/342(IMAPve_d_ORI_FS_OutOfFocus0) -> BusCreator/342  "IMAPve_d_ORI_FS_OutOfFocus0"
  Runnable_IMAP_10ms_sys/343(IMAPva_g_ORI_Obj_AbsAx) -> BusCreator/343  "IMAPva_g_ORI_Obj_AbsAx"
  Runnable_IMAP_10ms_sys/344(IMAPva_g_ORI_Obj_AbsAy) -> BusCreator/344  "IMAPva_g_ORI_Obj_AbsAy"
  Runnable_IMAP_10ms_sys/345(IMAPva_g_ORI_Obj_TTIPCStdDev) -> BusCreator/345  "IMAPva_g_ORI_Obj_TTIPCStdDev"
  Runnable_IMAP_10ms_sys/346(IMAPva_g_ORI_Obj_RelVely) -> BusCreator/346  "IMAPva_g_ORI_Obj_RelVely"
  Runnable_IMAP_10ms_sys/347(IMAPva_g_ORI_Obj_LateralDis) -> BusCreator/347  "IMAPva_g_ORI_Obj_LateralDis"
  Runnable_IMAP_10ms_sys/348(IMAPva_g_ORI_Obj_AbsAxStdDev) -> BusCreator/348  "IMAPva_g_ORI_Obj_AbsAxStdDev"
  Runnable_IMAP_10ms_sys/349(IMAPva_g_ORI_Obj_AbsAyStdDev) -> BusCreator/349  "IMAPva_g_ORI_Obj_AbsAyStdDev"
  Runnable_IMAP_10ms_sys/350(IMAPva_g_ORI_Obj_RelVelStdDev) -> BusCreator/350  "IMAPva_g_ORI_Obj_RelVelStdDev"
  Runnable_IMAP_10ms_sys/351(IMAPva_g_ORI_Obj_RelVelyStdDev) -> BusCreator/351  "IMAPva_g_ORI_Obj_RelVelyStdDev"
  Runnable_IMAP_10ms_sys/352(IMAPva_g_ORI_Obj_LongDisStdDev) -> BusCreator/352  "IMAPva_g_ORI_Obj_LongDisStdDev"
  Runnable_IMAP_10ms_sys/353(IMAPva_g_ORI_Obj_LateralDisStdDev) -> BusCreator/353  "IMAPva_g_ORI_Obj_LateralDisStdDev"
  Runnable_IMAP_10ms_sys/354(IMAPva_d_ORI_Obj_RelVelValid) -> BusCreator/354  "IMAPva_d_ORI_Obj_RelVelValid"
  Runnable_IMAP_10ms_sys/355(IMAPva_d_ORI_Obj_RelVelyValid) -> BusCreator/355  "IMAPva_d_ORI_Obj_RelVelyValid"
  Runnable_IMAP_10ms_sys/356(IMAPva_d_ORI_Obj_RelVelStdDevValid) -> BusCreator/356  "IMAPva_d_ORI_Obj_RelVelStdDevValid"
  Runnable_IMAP_10ms_sys/357(IMAPva_d_ORI_Obj_RelVelyStdDevValid) -> BusCreator/357  "IMAPva_d_ORI_Obj_RelVelyStdDevValid"
  Runnable_IMAP_10ms_sys/358(IMAPva_g_ORI_Obj_ExistProb) -> BusCreator/358  "IMAPva_g_ORI_Obj_ExistProb"
  Runnable_IMAP_10ms_sys/359(IMAPva_g_ORI_Obj_ClassProb) -> BusCreator/359  "IMAPva_g_ORI_Obj_ClassProb"
  Runnable_IMAP_10ms_sys/360(IMAPva_g_ORI_Obj_Height) -> BusCreator/360  "IMAPva_g_ORI_Obj_Height"
  Runnable_IMAP_10ms_sys/361(IMAPva_g_ORI_Obj_LengthStdDev) -> BusCreator/361  "IMAPva_g_ORI_Obj_LengthStdDev"
  Runnable_IMAP_10ms_sys/362(IMAPva_g_ORI_Obj_WidthStdDev) -> BusCreator/362  "IMAPva_g_ORI_Obj_WidthStdDev"
  Runnable_IMAP_10ms_sys/363(IMAPva_g_ORI_Obj_HeightStdDev) -> BusCreator/363  "IMAPva_g_ORI_Obj_HeightStdDev"
  Runnable_IMAP_10ms_sys/364(IMAPva_g_ORI_Obj_3DAngle) -> BusCreator/364  "IMAPva_g_ORI_Obj_3DAngle"
  Runnable_IMAP_10ms_sys/365(IMAPva_g_ORI_Obj_LAngleStdDev) -> BusCreator/365  "IMAPva_g_ORI_Obj_LAngleStdDev"
  Runnable_IMAP_10ms_sys/366(IMAPva_g_ORI_Obj_RAngleStdDev) -> BusCreator/366  "IMAPva_g_ORI_Obj_RAngleStdDev"
  Runnable_IMAP_10ms_sys/367(IMAPva_g_ORI_Obj_3DAngleStdDev) -> BusCreator/367  "IMAPva_g_ORI_Obj_3DAngleStdDev"
  Runnable_IMAP_10ms_sys/368(IMAPva_g_ORI_Obj_AngleRate) -> BusCreator/368  "IMAPva_g_ORI_Obj_AngleRate"
  Runnable_IMAP_10ms_sys/369(IMAPva_g_ORI_Obj_AngleRateStdDev) -> BusCreator/369  "IMAPva_g_ORI_Obj_AngleRateStdDev"
  Runnable_IMAP_10ms_sys/370(IMAPva_g_ORI_Obj_PhiBottom) -> BusCreator/370  "IMAPva_g_ORI_Obj_PhiBottom"
  Runnable_IMAP_10ms_sys/371(IMAPva_g_ORI_Obj_PhiBottomStdDev) -> BusCreator/371  "IMAPva_g_ORI_Obj_PhiBottomStdDev"
  Runnable_IMAP_10ms_sys/372(IMAPva_d_ORI_Obj_Measured) -> BusCreator/372  "IMAPva_d_ORI_Obj_Measured"
  Runnable_IMAP_10ms_sys/373(IMAPva_g_ORI_Obj_Heading) -> BusCreator/373  "IMAPva_g_ORI_Obj_Heading"
  Runnable_IMAP_10ms_sys/374(IMAPva_g_ORI_Obj_HeadingStdDev) -> BusCreator/374  "IMAPva_g_ORI_Obj_HeadingStdDev"
  Runnable_IMAP_10ms_sys/375(IMAPva_d_ORI_Obj_HeadOrientation) -> BusCreator/375  "IMAPva_d_ORI_Obj_HeadOrientation"
  Runnable_IMAP_10ms_sys/376(IMAPva_g_ORI_Obj_TTIPC) -> BusCreator/376  "IMAPva_g_ORI_Obj_TTIPC"
  Runnable_IMAP_10ms_sys/377(IMAPva_d_ORI_Obj_DirectionIndicator) -> BusCreator/377  "IMAPva_d_ORI_Obj_DirectionIndicator"
  Runnable_IMAP_10ms_sys/378(IMAPva_d_ORI_Obj_BrakeLight) -> BusCreator/378  "IMAPva_d_ORI_Obj_BrakeLight"
  Runnable_IMAP_10ms_sys/379(IMAPve_d_ORI_L0_ID) -> BusCreator/379  "IMAPve_d_ORI_L0_ID"
  Runnable_IMAP_10ms_sys/380(IMAPve_g_ORI_L0_ExistProb) -> BusCreator/380  "IMAPve_g_ORI_L0_ExistProb"
  Runnable_IMAP_10ms_sys/381(IMAPve_g_ORI_L0_DxStart) -> BusCreator/381  "IMAPve_g_ORI_L0_DxStart"
  Runnable_IMAP_10ms_sys/382(IMAPve_d_ORI_L0_ColorClass) -> BusCreator/382  "IMAPve_d_ORI_L0_ColorClass"
  Runnable_IMAP_10ms_sys/383(IMAPve_d_ORI_L0_MeasureType) -> BusCreator/383  "IMAPve_d_ORI_L0_MeasureType"
  Runnable_IMAP_10ms_sys/384(IMAPve_g_ORI_L0_TypeConf) -> BusCreator/384  "IMAPve_g_ORI_L0_TypeConf"
  Runnable_IMAP_10ms_sys/385(IMAPve_d_ORI_R0_ID) -> BusCreator/385  "IMAPve_d_ORI_R0_ID"
  Runnable_IMAP_10ms_sys/386(IMAPve_g_ORI_R0_ExistProb) -> BusCreator/386  "IMAPve_g_ORI_R0_ExistProb"
  Runnable_IMAP_10ms_sys/387(IMAPve_g_ORI_R0_Dxstart) -> BusCreator/387  "IMAPve_g_ORI_R0_Dxstart"
  Runnable_IMAP_10ms_sys/388(IMAPve_d_ORI_R0_ColorClass) -> BusCreator/388  "IMAPve_d_ORI_R0_ColorClass"
  Runnable_IMAP_10ms_sys/389(IMAPve_d_ORI_R0_MeasureType) -> BusCreator/389  "IMAPve_d_ORI_R0_MeasureType"
  Runnable_IMAP_10ms_sys/390(IMAPve_g_ORI_R0_TypeConf) -> BusCreator/390  "IMAPve_g_ORI_R0_TypeConf"
  Runnable_IMAP_10ms_sys/391(IMAPve_d_ORI_L1_ID) -> BusCreator/391  "IMAPve_d_ORI_L1_ID"
  Runnable_IMAP_10ms_sys/392(IMAPve_g_ORI_L1_ExistProb) -> BusCreator/392  "IMAPve_g_ORI_L1_ExistProb"
  Runnable_IMAP_10ms_sys/393(IMAPve_g_ORI_L1_Dxstart) -> BusCreator/393  "IMAPve_g_ORI_L1_Dxstart"
  Runnable_IMAP_10ms_sys/394(IMAPve_d_ORI_L1_ColorClass) -> BusCreator/394  "IMAPve_d_ORI_L1_ColorClass"
  Runnable_IMAP_10ms_sys/395(IMAPve_d_ORI_L1_MeasureType) -> BusCreator/395  "IMAPve_d_ORI_L1_MeasureType"
  Runnable_IMAP_10ms_sys/396(IMAPve_g_ORI_L1_TypeConf) -> BusCreator/396  "IMAPve_g_ORI_L1_TypeConf"
  Runnable_IMAP_10ms_sys/397(IMAPve_d_ORI_R1_ID) -> BusCreator/397  "IMAPve_d_ORI_R1_ID"
  Runnable_IMAP_10ms_sys/398(IMAPve_g_ORI_R1_ExistProb) -> BusCreator/398  "IMAPve_g_ORI_R1_ExistProb"
  Runnable_IMAP_10ms_sys/399(IMAPve_g_ORI_R1_Dxstart) -> BusCreator/399  "IMAPve_g_ORI_R1_Dxstart"
  Runnable_IMAP_10ms_sys/400(IMAPve_d_ORI_R1_ColorClass) -> BusCreator/400  "IMAPve_d_ORI_R1_ColorClass"
  Runnable_IMAP_10ms_sys/401(IMAPve_d_ORI_R1_MeasureType) -> BusCreator/401  "IMAPve_d_ORI_R1_MeasureType"
  Runnable_IMAP_10ms_sys/402(IMAPve_g_ORI_R1_TypeConf) -> BusCreator/402  "IMAPve_g_ORI_R1_TypeConf"
  Runnable_IMAP_10ms_sys/403(IMAPve_d_ORI_RoadedgeL0_ID) -> BusCreator/403  "IMAPve_d_ORI_RoadedgeL0_ID"
  Runnable_IMAP_10ms_sys/404(IMAPve_g_ORI_RoadedgeL0_ExistProb) -> BusCreator/404  "IMAPve_g_ORI_RoadedgeL0_ExistProb"
  Runnable_IMAP_10ms_sys/405(IMAPve_g_ORI_RoadedgeL0_DxStart) -> BusCreator/405  "IMAPve_g_ORI_RoadedgeL0_DxStart"
  Runnable_IMAP_10ms_sys/406(IMAPve_g_ORI_RoadedgeL0_DxEnd) -> BusCreator/406  "IMAPve_g_ORI_RoadedgeL0_DxEnd"
  Runnable_IMAP_10ms_sys/407(IMAPve_g_ORI_RoadedgeL0_C1) -> BusCreator/407  "IMAPve_g_ORI_RoadedgeL0_C1"
  Runnable_IMAP_10ms_sys/408(IMAPve_g_ORI_RoadedgeL0_C0) -> BusCreator/408  "IMAPve_g_ORI_RoadedgeL0_C0"
  Runnable_IMAP_10ms_sys/409(IMAPve_g_ORI_RoadedgeL0_C3) -> BusCreator/409  "IMAPve_g_ORI_RoadedgeL0_C3"
  Runnable_IMAP_10ms_sys/410(IMAPve_g_ORI_RoadedgeL0_C2) -> BusCreator/410  "IMAPve_g_ORI_RoadedgeL0_C2"
  Runnable_IMAP_10ms_sys/411(IMAPve_d_ORI_RoadedgeL0_MeasureType) -> BusCreator/411  "IMAPve_d_ORI_RoadedgeL0_MeasureType"
  Runnable_IMAP_10ms_sys/412(IMAPve_d_ORI_RoadedgeL0_Type) -> BusCreator/412  "IMAPve_d_ORI_RoadedgeL0_Type"
  Runnable_IMAP_10ms_sys/413(IMAPve_d_ORI_RoadedgeR0_ID) -> BusCreator/413  "IMAPve_d_ORI_RoadedgeR0_ID"
  Runnable_IMAP_10ms_sys/414(IMAPve_g_ORI_RoadedgeR0_ExistProb) -> BusCreator/414  "IMAPve_g_ORI_RoadedgeR0_ExistProb"
  Runnable_IMAP_10ms_sys/415(IMAPve_g_ORI_RoadedgeR0_DxStart) -> BusCreator/415  "IMAPve_g_ORI_RoadedgeR0_DxStart"
  Runnable_IMAP_10ms_sys/416(IMAPve_g_ORI_RoadedgeR0_DxEnd) -> BusCreator/416  "IMAPve_g_ORI_RoadedgeR0_DxEnd"
  Runnable_IMAP_10ms_sys/417(IMAPve_g_ORI_RoadedgeR0_C1) -> BusCreator/417  "IMAPve_g_ORI_RoadedgeR0_C1"
  Runnable_IMAP_10ms_sys/418(IMAPve_g_ORI_RoadedgeR0_C0) -> BusCreator/418  "IMAPve_g_ORI_RoadedgeR0_C0"
  Runnable_IMAP_10ms_sys/419(IMAPve_g_ORI_RoadedgeR0_C3) -> BusCreator/419  "IMAPve_g_ORI_RoadedgeR0_C3"
  Runnable_IMAP_10ms_sys/420(IMAPve_g_ORI_RoadedgeR0_C2) -> BusCreator/420  "IMAPve_g_ORI_RoadedgeR0_C2"
  Runnable_IMAP_10ms_sys/421(IMAPve_d_ORI_RoadedgeR0_MeasureType) -> BusCreator/421  "IMAPve_d_ORI_RoadedgeR0_MeasureType"
  Runnable_IMAP_10ms_sys/422(IMAPve_d_ORI_RoadedgeR0_Type) -> BusCreator/422  "IMAPve_d_ORI_RoadedgeR0_Type"
  Runnable_IMAP_10ms_sys/423(IMAPve_d_APA_AutoPark_WorkSt) -> BusCreator/423  "IMAPve_d_APA_AutoPark_WorkSt"
  Runnable_IMAP_10ms_sys/424(IMAPve_g_ob020H_100) -> BusCreator/424  "IMAPve_g_ob020H_100"
  Runnable_IMAP_10ms_sys/425(IMAPve_g_ob020L_100) -> BusCreator/425  "IMAPve_g_ob020L_100"
  Gain9/1 -> Data Type Conversion9/1
  Gain10/1 -> Data Type  Conversion75/1
  Gain11/1 -> Data Type  Conversion51/1
  Gain12/1 -> Data Type  Conversion50/1
  Bus Selector1/81 -> Runnable_IMAP_10ms_sys/171(SDFAve_g_Lrg_C0_BACK_COEF)  "<SDFAve_g_Lrg_C0_BACK_COEF (signal 95)>"
  Bus Selector1/82 -> Runnable_IMAP_10ms_sys/172(SDFAve_g_Lrg_C1_BACK_COEF)  "<SDFAve_g_Lrg_C1_BACK_COEF (signal 96)>"
  Bus Selector1/83 -> Runnable_IMAP_10ms_sys/173(SDFAve_g_Lrg_C2_BACK_COEF)  "<SDFAve_g_Lrg_C2_BACK_COEF (signal 97)>"
  Bus Selector1/84 -> Runnable_IMAP_10ms_sys/174(SDFAve_g_Lrg_C3_BACK_COEF)  "<SDFAve_g_Lrg_C3_BACK_COEF (signal 98)>"
  Bus Selector1/85 -> Runnable_IMAP_10ms_sys/175(SDFAve_g_Lrg_VIEW_RANGE_start)  "<SDFAve_g_Lrg_VIEW_RANGE_start (signal 99)>"
  Bus Selector1/86 -> Runnable_IMAP_10ms_sys/176(SDFAve_g_Lrg_VIEW_RANGE_end)  "<SDFAve_g_Lrg_VIEW_RANGE_end (signal 100)>"
  Bus Selector1/87 -> Runnable_IMAP_10ms_sys/177(SDFAve_y_Lrg_DETECT_QUALITY)  "<SDFAve_y_Lrg_DETECT_QUALITY (signal 109)>"
  Bus Selector1/88 -> Runnable_IMAP_10ms_sys/178(SDFAve_y_Lrg_LINE_TYPE)  "<SDFAve_y_Lrg_LINE_TYPE (signal 110)>"
  Bus Selector1/89 -> Runnable_IMAP_10ms_sys/179(SDFAve_g_Rrg_C0_BACK_COEF)  "<SDFAve_g_Rrg_C0_BACK_COEF (signal 101)>"
  Bus Selector1/90 -> Runnable_IMAP_10ms_sys/180(SDFAve_g_Rrg_C1_BACK_COEF)  "<SDFAve_g_Rrg_C1_BACK_COEF (signal 102)>"
  Bus Selector1/91 -> Runnable_IMAP_10ms_sys/181(SDFAve_g_Rrg_C2_BACK_COEF)  "<SDFAve_g_Rrg_C2_BACK_COEF (signal 103)>"
  Bus Selector1/92 -> Runnable_IMAP_10ms_sys/182(SDFAve_g_Rrg_C3_BACK_COEF)  "<SDFAve_g_Rrg_C3_BACK_COEF (signal 104)>"
  Bus Selector1/93 -> Runnable_IMAP_10ms_sys/183(SDFAve_g_Rrg_VIEW_RANGE_start)  "<SDFAve_g_Rrg_VIEW_RANGE_start (signal 105)>"
  Bus Selector1/94 -> Runnable_IMAP_10ms_sys/184(SDFAve_g_Rrg_VIEW_RANGE_end)  "<SDFAve_g_Rrg_VIEW_RANGE_end (signal 106)>"
  Bus Selector1/95 -> Runnable_IMAP_10ms_sys/185(SDFAve_y_Rrg_DETECT_QUALITY)  "<SDFAve_y_Rrg_DETECT_QUALITY (signal 107)>"
  Bus Selector1/96 -> Runnable_IMAP_10ms_sys/186(SDFAve_y_Rrg_LINE_TYPE)  "<SDFAve_y_Rrg_LINE_TYPE (signal 108)>"
  Manual Switch1/1 -> Runnable_IMAP_10ms_sys/187(SDFAve_y_ISAValue)
  Manual Switch2/1 -> Runnable_IMAP_10ms_sys/189(SDFAve_y_ISASignType)
  Bus Selector/4 -> Runnable_IMAP_10ms_sys/190(SDFAve_y_ISAStatus)  "<SDFAve_y_ISAStatus (signal 87)>"
  Bus Selector/5 -> Runnable_IMAP_10ms_sys/191(SDFAve_y_TSR_Sign_Type)  "<SDFAve_y_TSR_Sign_Type (signal 29)>"
  Bus Selector/6 -> Runnable_IMAP_10ms_sys/192(SDFAve_g_CameraSignalFault)  "<SDFAve_g_CameraSignalFault (signal 30)>"
  Bus Selector/7 -> Runnable_IMAP_10ms_sys/193(SDFAve_y_Radar_State)  "<SDFAve_y_Radar_State (signal 89)>"
  Bus Selector/8 -> Runnable_IMAP_10ms_sys/194(SDFAve_y_OperatingStatus)  "<SDFAve_y_OperatinfStatus (signal 90)>"
  Bus Selector/9 -> Runnable_IMAP_10ms_sys/195(SDFAve_y_Radar_FaultBitSetting_Signal)  "<SDFAve_y_Radar_FaultBitSetting_Signal (signal 94)>"
  Bus Selector/2 -> Runnable_IMAP_10ms_sys/188(SDFAve_y_ISAPopupMessage)  "<SDFAve_y_ISAPopupMessage (signal 88)>"
  Data Type Conversion13/1 -> Manual Switch1/1
  Read CM Dict18/1 -> Data Type Conversion13/1
  Bus Selector/1 -> Manual Switch1/2  "<SDFAve_y_ISAValue (signal 28)>"
  Bus Selector/3 -> Manual Switch2/2  "<SDFAve_y_ISASignType (signal 86)>"
  BCM_HazardSwitchSt/1 -> Runnable_IMAP_10ms_sys/39(SWINve_y_BCM_HazardSwitchrSt)
  MP5_HazardLampCtrlReq/1 -> Runnable_IMAP_10ms_sys/40(SWINve_y_MP5_HazardLampCtrlReq)
  TBOX_RemoteHazardReq/1 -> Runnable_IMAP_10ms_sys/41(SWINve_y_T_box_RemoteHazardReq)
  Data Type  Conversion32/1 -> Runnable_IMAP_10ms_sys/202(SWINve_y_EPS_SteeringAngle_Flag)  "EPS_SteeringAngle_Flag"
